simulink model "ForwardKinematic_YuMi"  (R2024a)
(part 20 of 23)

2903273033334964234439083875867/41538374868278621028243970633760768))/10384593717069655257060992658440192 + 34189201462609793352471527538206775118278208232606556159508725/57896044618658097711785492504343953926634992332820282019728792003956564819968))/9007199254740992))/1000 + (2436553109258773196144549622003023*cos(q6R)*(cos(q5R)*((7514214926474921*sin(q4R)*((7514214926474921*cos(q3R)*((7514214926474921*cos(q2R)*((398031123528767*cos(q1R))/562949953421312 - (1392340654334763*sin(q1R))/2251799813685248))/36893488147419103232 - (3480118470877607344838997022995*cos(q2R))/10141204801825835211973625643008 + sin(q2R)*((1392340654334763*cos(q1R))/2251799813685248 + (398031123528767*sin(q1R))/562949953421312)))/36893488147419103232 - sin(q3R)*((3480118470877607344838997022995*sin(q2R))/10141204801825835211973625643008 + cos(q2R)*((1392340654334763*cos(q1R))/2251799813685248 + (398031123528767*sin(q1R))/562949953421312) - (7514214926474921*sin(q2R)*((398031123528767*cos(q1R))/562949953421312 - (1392340654334763*sin(q1R))/2251799813685248))/36893488147419103232) + (9007199067919185*cos(q3R)*((3585145564851136108341178694895*cos(q1R))/5070602400912917605986812821504 - (12541089443950065443620820128155*sin(q1R))/20282409603651670423947251286016 + 2903273033334964234439083875867/41538374868278621028243970633760768))/9007199254740992))/36893488147419103232 + ((7514214926474921*cos(q4R))/36893488147419103232 + (4503599440548691*sin(q4R))/4503599627370496)*(cos(q3R)*((3480118470877607344838997022995*sin(q2R))/10141204801825835211973625643008 + cos(q2R)*((1392340654334763*cos(q1R))/2251799813685248 + (398031123528767*sin(q1R))/562949953421312) - (7514214926474921*sin(q2R)*((398031123528767*cos(q1R))/562949953421312 - (1392340654334763*sin(q1R))/2251799813685248))/36893488147419103232) + (7514214926474921*sin(q3R)*((7514214926474921*cos(q2R)*((398031123528767*cos(q1R))/562949953421312 - (1392340654334763*sin(q1R))/2251799813685248))/36893488147419103232 - (3480118470877607344838997022995*cos(q2R))/10141204801825835211973625643008 + sin(q2R)*((1392340654334763*cos(q1R))/2251799813685248 + (398031123528767*sin(q1R))/562949953421312)))/36893488147419103232 + (9007199067919185*sin(q3R)*((3585145564851136108341178694895*cos(q1R))/5070602400912917605986812821504 - (12541089443950065443620820128155*sin(q1R))/20282409603651670423947251286016 + 2903273033334964234439083875867/41538374868278621028243970633760768))/9007199254740992) - ((9007199067919185*cos(q4R))/9007199254740992 - (234819211581865*sin(q4R))/1152921504606846976)*((26939554316989768830159504461322709929728228295*cos(q1R))/187072209578355573530071658587684226515959365500928 + (31346119847137124244279794758002175024246659075*cos(q2R))/91343852333181432387730302044767688728495783936 - (94236441493986648894942587121893377357613500755*sin(q1R))/748288838313422294120286634350736906063837462003712 - (67682029681889335677290557259385*cos(q2R)*((398031123528767*cos(q1R))/562949953421312 - (1392340654334763*sin(q1R))/2251799813685248))/332306998946228968225951765070086144 - (9007199067919185*sin(q2R)*((1392340654334763*cos(q1R))/2251799813685248 + (398031123528767*sin(q1R))/562949953421312))/9007199254740992 + 21815817562717709140362801846989786744252631507/1532495540865888858358347027150309183618739122183602176)) - (7514214926474921*sin(q5R)*(((4503599440548691*cos(q4R))/4503599627370496 - (7514214926474921*sin(q4R))/36893488147419103232)*(cos(q3R)*((3480118470877607344838997022995*sin(q2R))/10141204801825835211973625643008 + cos(q2R)*((1392340654334763*cos(q1R))/2251799813685248 + (398031123528767*sin(q1R))/562949953421312) - (7514214926474921*sin(q2R)*((398031123528767*cos(q1R))/562949953421312 - (1392340654334763*sin(q1R))/2251799813685248))/36893488147419103232) + (7514214926474921*sin(q3R)*((7514214926474921*cos(q2R)*((398031123528767*cos(q1R))/562949953421312 - (1392340654334763*sin(q1R))/2251799813685248))/36893488147419103232 - (3480118470877607344838997022995*cos(q2R))/10141204801825835211973625643008 + sin(q2R)*((1392340654334763*cos(q1R))/2251799813685248 + (398031123528767*sin(q1R))/562949953421312)))/36893488147419103232 + (9007199067919185*sin(q3R)*((3585145564851136108341178694895*cos(q1R))/5070602400912917605986812821504 - (12541089443950065443620820128155*sin(q1R))/20282409603651670423947251286016 + 2903273033334964234439083875867/41538374868278621028243970633760768))/9007199254740992) + ((234819211581865*cos(q4R))/1152921504606846976 + (9007199067919185*sin(q4R))/9007199254740992)*((26939554316989768830159504461322709929728228295*cos(q1R))/187072209578355573530071658587684226515959365500928 + (31346119847137124244279794758002175024246659075*cos(q2R))/91343852333181432387730302044767688728495783936 - (94236441493986648894942587121893377357613500755*sin(q1R))/748288838313422294120286634350736906063837462003712 - (67682029681889335677290557259385*cos(q2R)*((398031123528767*cos(q1R))/562949953421312 - (1392340654334763*sin(q1R))/2251799813685248))/332306998946228968225951765070086144 - (9007199067919185*sin(q2R)*((1392340654334763*cos(q1R))/2251799813685248 + (398031123528767*sin(q1R))/562949953421312))/9007199254740992 + 21815817562717709140362801846989786744252631507/1532495540865888858358347027150309183618739122183602176) + (7514214926474921*cos(q4R)*((7514214926474921*cos(q3R)*((7514214926474921*cos(q2R)*((398031123528767*cos(q1R))/562949953421312 - (1392340654334763*sin(q1R))/2251799813685248))/36893488147419103232 - (3480118470877607344838997022995*cos(q2R))/10141204801825835211973625643008 + sin(q2R)*((1392340654334763*cos(q1R))/2251799813685248 + (398031123528767*sin(q1R))/562949953421312)))/36893488147419103232 - sin(q3R)*((3480118470877607344838997022995*sin(q2R))/10141204801825835211973625643008 + cos(q2R)*((1392340654334763*cos(q1R))/2251799813685248 + (398031123528767*sin(q1R))/562949953421312) - (7514214926474921*sin(q2R)*((398031123528767*cos(q1R))/562949953421312 - (1392340654334763*sin(q1R))/2251799813685248))/36893488147419103232) + (9007199067919185*cos(q3R)*((3585145564851136108341178694895*cos(q1R))/5070602400912917605986812821504 - (12541089443950065443620820128155*sin(q1R))/20282409603651670423947251286016 + 2903273033334964234439083875867/41538374868278621028243970633760768))/9007199254740992))/36893488147419103232))/36893488147419103232 + (9007199067919185*sin(q5R)*((42218993040650622024393554167529407181397382817729417611526625*cos(q1R))/7067388259113537318333190002971674063309935587502475832486424805170479104 + (49124851885283889459147163519037433596494512994900179139213125*cos(q2R))/3450873173395281893717377931138512726225554486085193277581262111899648 - (147684984717849177105467939785270041851792306559769220895307125*sin(q1R))/28269553036454149273332760011886696253239742350009903329945699220681916416 - (67682029681889335677290557259385*cos(q3R)*((7514214926474921*cos(q2R)*((398031123528767*cos(q1R))/562949953421312 - (1392340654334763*sin(q1R))/2251799813685248))/36893488147419103232 - (3480118470877607344838997022995*cos(q2R))/10141204801825835211973625643008 + sin(q2R)*((1392340654334763*cos(q1R))/2251799813685248 + (398031123528767*sin(q1R))/562949953421312)))/332306998946228968225951765070086144 + (234819211581865*cos(q3R)*((3480118470877607344838997022995*sin(q2R))/10141204801825835211973625643008 + cos(q2R)*((1392340654334763*cos(q1R))/2251799813685248 + (398031123528767*sin(q1R))/562949953421312) - (7514214926474921*sin(q2R)*((398031123528767*cos(q1R))/562949953421312 - (1392340654334763*sin(q1R))/2251799813685248))/36893488147419103232))/1152921504606846976 + (1764482024691522628700660907665*sin(q3R)*((7514214926474921*cos(q2R)*((398031123528767*cos(q1R))/562949953421312 - (1392340654334763*sin(q1R))/2251799813685248))/36893488147419103232 - (3480118470877607344838997022995*cos(q2R))/10141204801825835211973625643008 + sin(q2R)*((1392340654334763*cos(q1R))/2251799813685248 + (398031123528767*sin(q1R))/562949953421312)))/42535295865117307932921825928971026432 + (9007199067919185*sin(q3R)*((3480118470877607344838997022995*sin(q2R))/10141204801825835211973625643008 + cos(q2R)*((1392340654334763*cos(q1R))/2251799813685248 + (398031123528767*sin(q1R))/562949953421312) - (7514214926474921*sin(q2R)*((398031123528767*cos(q1R))/562949953421312 - (1392340654334763*sin(q1R))/2251799813685248))/36893488147419103232))/9007199254740992 - (106069577339469832923929692356850887620017617375*cos(q2R)*((398031123528767*cos(q1R))/562949953421312 - (1392340654334763*sin(q1R))/2251799813685248))/12554203470773361527671578846415332832204710888928069025792 - (81129635049124235038645691064225*cos(q3R)*((3585145564851136108341178694895*cos(q1R))/5070602400912917605986812821504 - (12541089443950065443620820128155*sin(q1R))/20282409603651670423947251286016 + 2903273033334964234439083875867/41538374868278621028243970633760768))/81129638414606681695789005144064 - (14115856197532180673579726082375*sin(q2R)*((1392340654334763*cos(q1R))/2251799813685248 + (398031123528767*sin(q1R))/562949953421312))/340282366920938463463374607431768211456 + (2115063383689692319117831580025*sin(q3R)*((3585145564851136108341178694895*cos(q1R))/5070602400912917605986812821504 - (12541089443950065443620820128155*sin(q1R))/20282409603651670423947251286016 + 2903273033334964234439083875867/41538374868278621028243970633760768))/10384593717069655257060992658440192 + 34189201462609793352471527538206775118278208232606556159508725/57896044618658097711785492504343953926634992332820282019728792003956564819968))/9007199254740992))/332306998946228968225951765070086144000 + (324259171862923063*sin(q6R)*((7514214926474921*cos(q5R)*(((4503599440548691*cos(q4R))/4503599627370496 - (7514214926474921*sin(q4R))/36893488147419103232)*(cos(q3R)*((3480118470877607344838997022995*sin(q2R))/10141204801825835211973625643008 + cos(q2R)*((1392340654334763*cos(q1R))/2251799813685248 + (398031123528767*sin(q1R))/562949953421312) - (7514214926474921*sin(q2R)*((398031123528767*cos(q1R))/562949953421312 - (1392340654334763*sin(q1R))/2251799813685248))/36893488147419103232) + (7514214926474921*sin(q3R)*((7514214926474921*cos(q2R)*((398031123528767*cos(q1R))/562949953421312 - (1392340654334763*sin(q1R))/2251799813685248))/36893488147419103232 - (3480118470877607344838997022995*cos(q2R))/10141204801825835211973625643008 + sin(q2R)*((1392340654334763*cos(q1R))/2251799813685248 + (398031123528767*sin(q1R))/562949953421312)))/36893488147419103232 + (9007199067919185*sin(q3R)*((3585145564851136108341178694895*cos(q1R))/5070602400912917605986812821504 - (12541089443950065443620820128155*sin(q1R))/20282409603651670423947251286016 + 2903273033334964234439083875867/41538374868278621028243970633760768))/9007199254740992) + ((234819211581865*cos(q4R))/1152921504606846976 + (9007199067919185*sin(q4R))/9007199254740992)*((26939554316989768830159504461322709929728228295*cos(q1R))/187072209578355573530071658587684226515959365500928 + (31346119847137124244279794758002175024246659075*cos(q2R))/91343852333181432387730302044767688728495783936 - (94236441493986648894942587121893377357613500755*sin(q1R))/748288838313422294120286634350736906063837462003712 - (67682029681889335677290557259385*cos(q2R)*((398031123528767*cos(q1R))/562949953421312 - (1392340654334763*sin(q1R))/2251799813685248))/332306998946228968225951765070086144 - (9007199067919185*sin(q2R)*((1392340654334763*cos(q1R))/2251799813685248 + (398031123528767*sin(q1R))/562949953421312))/9007199254740992 + 21815817562717709140362801846989786744252631507/1532495540865888858358347027150309183618739122183602176) + (7514214926474921*cos(q4R)*((7514214926474921*cos(q3R)*((7514214926474921*cos(q2R)*((398031123528767*cos(q1R))/562949953421312 - (1392340654334763*sin(q1R))/2251799813685248))/36893488147419103232 - (3480118470877607344838997022995*cos(q2R))/10141204801825835211973625643008 + sin(q2R)*((1392340654334763*cos(q1R))/2251799813685248 + (398031123528767*sin(q1R))/562949953421312)))/36893488147419103232 - sin(q3R)*((3480118470877607344838997022995*sin(q2R))/10141204801825835211973625643008 + cos(q2R)*((1392340654334763*cos(q1R))/2251799813685248 + (398031123528767*sin(q1R))/562949953421312) - (7514214926474921*sin(q2R)*((398031123528767*cos(q1R))/562949953421312 - (1392340654334763*sin(q1R))/2251799813685248))/36893488147419103232) + (9007199067919185*cos(q3R)*((3585145564851136108341178694895*cos(q1R))/5070602400912917605986812821504 - (12541089443950065443620820128155*sin(q1R))/20282409603651670423947251286016 + 2903273033334964234439083875867/41538374868278621028243970633760768))/9007199254740992))/36893488147419103232))/36893488147419103232 + sin(q5R)*((7514214926474921*sin(q4R)*((7514214926474921*cos(q3R)*((7514214926474921*cos(q2R)*((398031123528767*cos(q1R))/562949953421312 - (1392340654334763*sin(q1R))/2251799813685248))/36893488147419103232 - (3480118470877607344838997022995*cos(q2R))/10141204801825835211973625643008 + sin(q2R)*((1392340654334763*cos(q1R))/2251799813685248 + (398031123528767*sin(q1R))/562949953421312)))/36893488147419103232 - sin(q3R)*((3480118470877607344838997022995*sin(q2R))/10141204801825835211973625643008 + cos(q2R)*((1392340654334763*cos(q1R))/2251799813685248 + (398031123528767*sin(q1R))/562949953421312) - (7514214926474921*sin(q2R)*((398031123528767*cos(q1R))/562949953421312 - (1392340654334763*sin(q1R))/2251799813685248))/36893488147419103232) + (9007199067919185*cos(q3R)*((3585145564851136108341178694895*cos(q1R))/5070602400912917605986812821504 - (12541089443950065443620820128155*sin(q1R))/20282409603651670423947251286016 + 2903273033334964234439083875867/41538374868278621028243970633760768))/9007199254740992))/36893488147419103232 + ((7514214926474921*cos(q4R))/36893488147419103232 + (4503599440548691*sin(q4R))/4503599627370496)*(cos(q3R)*((3480118470877607344838997022995*sin(q2R))/10141204801825835211973625643008 + cos(q2R)*((1392340654334763*cos(q1R))/2251799813685248 + (398031123528767*sin(q1R))/562949953421312) - (7514214926474921*sin(q2R)*((398031123528767*cos(q1R))/562949953421312 - (1392340654334763*sin(q1R))/2251799813685248))/36893488147419103232) + (7514214926474921*sin(q3R)*((7514214926474921*cos(q2R)*((398031123528767*cos(q1R))/562949953421312 - (1392340654334763*sin(q1R))/2251799813685248))/36893488147419103232 - (3480118470877607344838997022995*cos(q2R))/10141204801825835211973625643008 + sin(q2R)*((1392340654334763*cos(q1R))/2251799813685248 + (398031123528767*sin(q1R))/562949953421312)))/36893488147419103232 + (9007199067919185*sin(q3R)*((3585145564851136108341178694895*cos(q1R))/5070602400912917605986812821504 - (12541089443950065443620820128155*sin(q1R))/20282409603651670423947251286016 + 2903273033334964234439083875867/41538374868278621028243970633760768))/9007199254740992) - ((9007199067919185*cos(q4R))/9007199254740992 - (234819211581865*sin(q4R))/1152921504606846976)*((26939554316989768830159504461322709929728228295*cos(q1R))/187072209578355573530071658587684226515959365500928 + (31346119847137124244279794758002175024246659075*cos(q2R))/91343852333181432387730302044767688728495783936 - (94236441493986648894942587121893377357613500755*sin(q1R))/748288838313422294120286634350736906063837462003712 - (67682029681889335677290557259385*cos(q2R)*((398031123528767*cos(q1R))/562949953421312 - (1392340654334763*sin(q1R))/2251799813685248))/332306998946228968225951765070086144 - (9007199067919185*sin(q2R)*((1392340654334763*cos(q1R))/2251799813685248 + (398031123528767*sin(q1R))/562949953421312))/9007199254740992 + 21815817562717709140362801846989786744252631507/1532495540865888858358347027150309183618739122183602176)) - (9007199067919185*cos(q5R)*((42218993040650622024393554167529407181397382817729417611526625*cos(q1R))/7067388259113537318333190002971674063309935587502475832486424805170479104 + (49124851885283889459147163519037433596494512994900179139213125*cos(q2R))/3450873173395281893717377931138512726225554486085193277581262111899648 - (147684984717849177105467939785270041851792306559769220895307125*sin(q1R))/28269553036454149273332760011886696253239742350009903329945699220681916416 - (67682029681889335677290557259385*cos(q3R)*((7514214926474921*cos(q2R)*((398031123528767*cos(q1R))/562949953421312 - (1392340654334763*sin(q1R))/2251799813685248))/36893488147419103232 - (3480118470877607344838997022995*cos(q2R))/10141204801825835211973625643008 + sin(q2R)*((1392340654334763*cos(q1R))/2251799813685248 + (398031123528767*sin(q1R))/562949953421312)))/332306998946228968225951765070086144 + (234819211581865*cos(q3R)*((3480118470877607344838997022995*sin(q2R))/10141204801825835211973625643008 + cos(q2R)*((1392340654334763*cos(q1R))/2251799813685248 + (398031123528767*sin(q1R))/562949953421312) - (7514214926474921*sin(q2R)*((398031123528767*cos(q1R))/562949953421312 - (1392340654334763*sin(q1R))/2251799813685248))/36893488147419103232))/1152921504606846976 + (1764482024691522628700660907665*sin(q3R)*((7514214926474921*cos(q2R)*((398031123528767*cos(q1R))/562949953421312 - (1392340654334763*sin(q1R))/2251799813685248))/36893488147419103232 - (3480118470877607344838997022995*cos(q2R))/10141204801825835211973625643008 + sin(q2R)*((1392340654334763*cos(q1R))/2251799813685248 + (398031123528767*sin(q1R))/562949953421312)))/42535295865117307932921825928971026432 + (9007199067919185*sin(q3R)*((3480118470877607344838997022995*sin(q2R))/10141204801825835211973625643008 + cos(q2R)*((1392340654334763*cos(q1R))/2251799813685248 + (398031123528767*sin(q1R))/562949953421312) - (7514214926474921*sin(q2R)*((398031123528767*cos(q1R))/562949953421312 - (1392340654334763*sin(q1R))/2251799813685248))/36893488147419103232))/9007199254740992 - (106069577339469832923929692356850887620017617375*cos(q2R)*((398031123528767*cos(q1R))/562949953421312 - (1392340654334763*sin(q1R))/2251799813685248))/12554203470773361527671578846415332832204710888928069025792 - (81129635049124235038645691064225*cos(q3R)*((3585145564851136108341178694895*cos(q1R))/5070602400912917605986812821504 - (12541089443950065443620820128155*sin(q1R))/20282409603651670423947251286016 + 2903273033334964234439083875867/41538374868278621028243970633760768))/81129638414606681695789005144064 - (14115856197532180673579726082375*sin(q2R)*((1392340654334763*cos(q1R))/2251799813685248 + (398031123528767*sin(q1R))/562949953421312))/340282366920938463463374607431768211456 + (2115063383689692319117831580025*sin(q3R)*((3585145564851136108341178694895*cos(q1R))/5070602400912917605986812821504 - (12541089443950065443620820128155*sin(q1R))/20282409603651670423947251286016 + 2903273033334964234439083875867/41538374868278621028243970633760768))/10384593717069655257060992658440192 + 34189201462609793352471527538206775118278208232606556159508725/57896044618658097711785492504343953926634992332820282019728792003956564819968))/9007199254740992))/9007199254740992000 + (712008244765680093343103025701132101054572137019*sin(q5R)*(((4503599440548691*cos(q4R))/4503599627370496 - (7514214926474921*sin(q4R))/36893488147419103232)*(cos(q3R)*((3480118470877607344838997022995*sin(q2R))/10141204801825835211973625643008 + cos(q2R)*((1392340654334763*cos(q1R))/2251799813685248 + (398031123528767*sin(q1R))/562949953421312) - (7514214926474921*sin(q2R)*((398031123528767*cos(q1R))/562949953421312 - (1392340654334763*sin(q1R))/2251799813685248))/36893488147419103232) + (7514214926474921*sin(q3R)*((7514214926474921*cos(q2R)*((398031123528767*cos(q1R))/562949953421312 - (1392340654334763*sin(q1R))/2251799813685248))/36893488147419103232 - (3480118470877607344838997022995*cos(q2R))/10141204801825835211973625643008 + sin(q2R)*((1392340654334763*cos(q1R))/2251799813685248 + (398031123528767*sin(q1R))/562949953421312)))/36893488147419103232 + (9007199067919185*sin(q3R)*((3585145564851136108341178694895*cos(q1R))/5070602400912917605986812821504 - (12541089443950065443620820128155*sin(q1R))/20282409603651670423947251286016 + 2903273033334964234439083875867/41538374868278621028243970633760768))/9007199254740992) + ((234819211581865*cos(q4R))/1152921504606846976 + (9007199067919185*sin(q4R))/9007199254740992)*((26939554316989768830159504461322709929728228295*cos(q1R))/187072209578355573530071658587684226515959365500928 + (31346119847137124244279794758002175024246659075*cos(q2R))/91343852333181432387730302044767688728495783936 - (94236441493986648894942587121893377357613500755*sin(q1R))/748288838313422294120286634350736906063837462003712 - (67682029681889335677290557259385*cos(q2R)*((398031123528767*cos(q1R))/562949953421312 - (1392340654334763*sin(q1R))/2251799813685248))/332306998946228968225951765070086144 - (9007199067919185*sin(q2R)*((1392340654334763*cos(q1R))/2251799813685248 + (398031123528767*sin(q1R))/562949953421312))/9007199254740992 + 21815817562717709140362801846989786744252631507/1532495540865888858358347027150309183618739122183602176) + (7514214926474921*cos(q4R)*((7514214926474921*cos(q3R)*((7514214926474921*cos(q2R)*((398031123528767*cos(q1R))/562949953421312 - (1392340654334763*sin(q1R))/2251799813685248))/36893488147419103232 - (3480118470877607344838997022995*cos(q2R))/10141204801825835211973625643008 + sin(q2R)*((1392340654334763*cos(q1R))/2251799813685248 + (398031123528767*sin(q1R))/562949953421312)))/36893488147419103232 - sin(q3R)*((3480118470877607344838997022995*sin(q2R))/10141204801825835211973625643008 + cos(q2R)*((1392340654334763*cos(q1R))/2251799813685248 + (398031123528767*sin(q1R))/562949953421312) - (7514214926474921*sin(q2R)*((398031123528767*cos(q1R))/562949953421312 - (1392340654334763*sin(q1R))/2251799813685248))/36893488147419103232) + (9007199067919185*cos(q3R)*((3585145564851136108341178694895*cos(q1R))/5070602400912917605986812821504 - (12541089443950065443620820128155*sin(q1R))/20282409603651670423947251286016 + 2903273033334964234439083875867/41538374868278621028243970633760768))/9007199254740992))/36893488147419103232))/2451992865385422173373355243440494693789982595493763481600 - (94754841554645069948206780163139*cos(q5R)*((7514214926474921*sin(q4R)*((7514214926474921*cos(q3R)*((7514214926474921*cos(q2R)*((398031123528767*cos(q1R))/562949953421312 - (1392340654334763*sin(q1R))/2251799813685248))/36893488147419103232 - (3480118470877607344838997022995*cos(q2R))/10141204801825835211973625643008 + sin(q2R)*((1392340654334763*cos(q1R))/2251799813685248 + (398031123528767*sin(q1R))/562949953421312)))/36893488147419103232 - sin(q3R)*((3480118470877607344838997022995*sin(q2R))/10141204801825835211973625643008 + cos(q2R)*((1392340654334763*cos(q1R))/2251799813685248 + (398031123528767*sin(q1R))/562949953421312) - (7514214926474921*sin(q2R)*((398031123528767*cos(q1R))/562949953421312 - (1392340654334763*sin(q1R))/2251799813685248))/36893488147419103232) + (9007199067919185*cos(q3R)*((3585145564851136108341178694895*cos(q1R))/5070602400912917605986812821504 - (12541089443950065443620820128155*sin(q1R))/20282409603651670423947251286016 + 2903273033334964234439083875867/41538374868278621028243970633760768))/9007199254740992))/36893488147419103232 + ((7514214926474921*cos(q4R))/36893488147419103232 + (4503599440548691*sin(q4R))/4503599627370496)*(cos(q3R)*((3480118470877607344838997022995*sin(q2R))/10141204801825835211973625643008 + cos(q2R)*((1392340654334763*cos(q1R))/2251799813685248 + (398031123528767*sin(q1R))/562949953421312) - (7514214926474921*sin(q2R)*((398031123528767*cos(q1R))/562949953421312 - (1392340654334763*sin(q1R))/2251799813685248))/36893488147419103232) + (7514214926474921*sin(q3R)*((7514214926474921*cos(q2R)*((398031123528767*cos(q1R))/562949953421312 - (1392340654334763*sin(q1R))/2251799813685248))/36893488147419103232 - (3480118470877607344838997022995*cos(q2R))/10141204801825835211973625643008 + sin(q2R)*((1392340654334763*cos(q1R))/2251799813685248 + (398031123528767*sin(q1R))/562949953421312)))/36893488147419103232 + (9007199067919185*sin(q3R)*((3585145564851136108341178694895*cos(q1R))/5070602400912917605986812821504 - (12541089443950065443620820128155*sin(q1R))/20282409603651670423947251286016 + 2903273033334964234439083875867/41538374868278621028243970633760768))/9007199254740992) - ((9007199067919185*cos(q4R))/9007199254740992 - (234819211581865*sin(q4R))/1152921504606846976)*((26939554316989768830159504461322709929728228295*cos(q1R))/187072209578355573530071658587684226515959365500928 + (31346119847137124244279794758002175024246659075*cos(q2R))/91343852333181432387730302044767688728495783936 - (94236441493986648894942587121893377357613500755*sin(q1R))/748288838313422294120286634350736906063837462003712 - (67682029681889335677290557259385*cos(q2R)*((398031123528767*cos(q1R))/562949953421312 - (1392340654334763*sin(q1R))/2251799813685248))/332306998946228968225951765070086144 - (9007199067919185*sin(q2R)*((1392340654334763*cos(q1R))/2251799813685248 + (398031123528767*sin(q1R))/562949953421312))/9007199254740992 + 21815817562717709140362801846989786744252631507/1532495540865888858358347027150309183618739122183602176)))/66461399789245793645190353014017228800 + (202883803014822867*sin(q6R)*(cos(q5R)*((7514214926474921*sin(q4R)*((7514214926474921*cos(q3R)*((7514214926474921*cos(q2R)*((398031123528767*cos(q1R))/562949953421312 - (1392340654334763*sin(q1R))/2251799813685248))/36893488147419103232 - (3480118470877607344838997022995*cos(q2R))/10141204801825835211973625643008 + sin(q2R)*((1392340654334763*cos(q1R))/2251799813685248 + (398031123528767*sin(q1R))/562949953421312)))/36893488147419103232 - sin(q3R)*((3480118470877607344838997022995*sin(q2R))/10141204801825835211973625643008 + cos(q2R)*((1392340654334763*cos(q1R))/2251799813685248 + (398031123528767*sin(q1R))/562949953421312) - (7514214926474921*sin(q2R)*((398031123528767*cos(q1R))/562949953421312 - (1392340654334763*sin(q1R))/2251799813685248))/36893488147419103232) + (9007199067919185*cos(q3R)*((3585145564851136108341178694895*cos(q1R))/5070602400912917605986812821504 - (12541089443950065443620820128155*sin(q1R))/20282409603651670423947251286016 + 2903273033334964234439083875867/41538374868278621028243970633760768))/9007199254740992))/36893488147419103232 + ((7514214926474921*cos(q4R))/36893488147419103232 + (4503599440548691*sin(q4R))/4503599627370496)*(cos(q3R)*((3480118470877607344838997022995*sin(q2R))/10141204801825835211973625643008 + cos(q2R)*((1392340654334763*cos(q1R))/2251799813685248 + (398031123528767*sin(q1R))/562949953421312) - (7514214926474921*sin(q2R)*((398031123528767*cos(q1R))/562949953421312 - (1392340654334763*sin(q1R))/2251799813685248))/36893488147419103232) + (7514214926474921*sin(q3R)*((7514214926474921*cos(q2R)*((398031123528767*cos(q1R))/562949953421312 - (1392340654334763*sin(q1R))/2251799813685248))/36893488147419103232 - (3480118470877607344838997022995*cos(q2R))/10141204801825835211973625643008 + sin(q2R)*((1392340654334763*cos(q1R))/2251799813685248 + (398031123528767*sin(q1R))/562949953421312)))/36893488147419103232 + (9007199067919185*sin(q3R)*((3585145564851136108341178694895*cos(q1R))/5070602400912917605986812821504 - (12541089443950065443620820128155*sin(q1R))/20282409603651670423947251286016 + 2903273033334964234439083875867/41538374868278621028243970633760768))/9007199254740992) - ((9007199067919185*cos(q4R))/9007199254740992 - (234819211581865*sin(q4R))/1152921504606846976)*((26939554316989768830159504461322709929728228295*cos(q1R))/187072209578355573530071658587684226515959365500928 + (31346119847137124244279794758002175024246659075*cos(q2R))/91343852333181432387730302044767688728495783936 - (94236441493986648894942587121893377357613500755*sin(q1R))/748288838313422294120286634350736906063837462003712 - (67682029681889335677290557259385*cos(q2R)*((398031123528767*cos(q1R))/562949953421312 - (1392340654334763*sin(q1R))/2251799813685248))/332306998946228968225951765070086144 - (9007199067919185*sin(q2R)*((1392340654334763*cos(q1R))/2251799813685248 + (398031123528767*sin(q1R))/562949953421312))/9007199254740992 + 21815817562717709140362801846989786744252631507/1532495540865888858358347027150309183618739122183602176)) - (7514214926474921*sin(q5R)*(((4503599440548691*cos(q4R))/4503599627370496 - (7514214926474921*sin(q4R))/36893488147419103232)*(cos(q3R)*((3480118470877607344838997022995*sin(q2R))/10141204801825835211973625643008 + cos(q2R)*((1392340654334763*cos(q1R))/2251799813685248 + (398031123528767*sin(q1R))/562949953421312) - (7514214926474921*sin(q2R)*((398031123528767*cos(q1R))/562949953421312 - (1392340654334763*sin(q1R))/2251799813685248))/36893488147419103232) + (7514214926474921*sin(q3R)*((7514214926474921*cos(q2R)*((398031123528767*cos(q1R))/562949953421312 - (1392340654334763*sin(q1R))/2251799813685248))/36893488147419103232 - (3480118470877607344838997022995*cos(q2R))/10141204801825835211973625643008 + sin(q2R)*((1392340654334763*cos(q1R))/2251799813685248 + (398031123528767*sin(q1R))/562949953421312)))/36893488147419103232 + (9007199067919185*sin(q3R)*((3585145564851136108341178694895*cos(q1R))/5070602400912917605986812821504 - (12541089443950065443620820128155*sin(q1R))/20282409603651670423947251286016 + 2903273033334964234439083875867/41538374868278621028243970633760768))/9007199254740992) + ((234819211581865*cos(q4R))/1152921504606846976 + (9007199067919185*sin(q4R))/9007199254740992)*((26939554316989768830159504461322709929728228295*cos(q1R))/187072209578355573530071658587684226515959365500928 + (31346119847137124244279794758002175024246659075*cos(q2R))/91343852333181432387730302044767688728495783936 - (94236441493986648894942587121893377357613500755*sin(q1R))/748288838313422294120286634350736906063837462003712 - (67682029681889335677290557259385*cos(q2R)*((398031123528767*cos(q1R))/562949953421312 - (1392340654334763*sin(q1R))/2251799813685248))/332306998946228968225951765070086144 - (9007199067919185*sin(q2R)*((1392340654334763*cos(q1R))/2251799813685248 + (398031123528767*sin(q1R))/562949953421312))/9007199254740992 + 21815817562717709140362801846989786744252631507/1532495540865888858358347027150309183618739122183602176) + (7514214926474921*cos(q4R)*((7514214926474921*cos(q3R)*((7514214926474921*cos(q2R)*((398031123528767*cos(q1R))/562949953421312 - (1392340654334763*sin(q1R))/2251799813685248))/36893488147419103232 - (3480118470877607344838997022995*cos(q2R))/10141204801825835211973625643008 + sin(q2R)*((1392340654334763*cos(q1R))/2251799813685248 + (398031123528767*sin(q1R))/562949953421312)))/36893488147419103232 - sin(q3R)*((3480118470877607344838997022995*sin(q2R))/10141204801825835211973625643008 + cos(q2R)*((1392340654334763*cos(q1R))/2251799813685248 + (398031123528767*sin(q1R))/562949953421312) - (7514214926474921*sin(q2R)*((398031123528767*cos(q1R))/562949953421312 - (1392340654334763*sin(q1R))/2251799813685248))/36893488147419103232) + (9007199067919185*cos(q3R)*((3585145564851136108341178694895*cos(q1R))/5070602400912917605986812821504 - (12541089443950065443620820128155*sin(q1R))/20282409603651670423947251286016 + 2903273033334964234439083875867/41538374868278621028243970633760768))/9007199254740992))/36893488147419103232))/36893488147419103232 + (9007199067919185*sin(q5R)*((42218993040650622024393554167529407181397382817729417611526625*cos(q1R))/7067388259113537318333190002971674063309935587502475832486424805170479104 + (49124851885283889459147163519037433596494512994900179139213125*cos(q2R))/3450873173395281893717377931138512726225554486085193277581262111899648 - (147684984717849177105467939785270041851792306559769220895307125*sin(q1R))/28269553036454149273332760011886696253239742350009903329945699220681916416 - (67682029681889335677290557259385*cos(q3R)*((7514214926474921*cos(q2R)*((398031123528767*cos(q1R))/562949953421312 - (1392340654334763*sin(q1R))/2251799813685248))/36893488147419103232 - (3480118470877607344838997022995*cos(q2R))/10141204801825835211973625643008 + sin(q2R)*((1392340654334763*cos(q1R))/2251799813685248 + (398031123528767*sin(q1R))/562949953421312)))/332306998946228968225951765070086144 + (234819211581865*cos(q3R)*((3480118470877607344838997022995*sin(q2R))/10141204801825835211973625643008 + cos(q2R)*((1392340654334763*cos(q1R))/2251799813685248 + (398031123528767*sin(q1R))/562949953421312) - (7514214926474921*sin(q2R)*((398031123528767*cos(q1R))/562949953421312 - (1392340654334763*sin(q1R))/2251799813685248))/36893488147419103232))/1152921504606846976 + (1764482024691522628700660907665*sin(q3R)*((7514214926474921*cos(q2R)*((398031123528767*cos(q1R))/562949953421312 - (1392340654334763*sin(q1R))/2251799813685248))/36893488147419103232 - (3480118470877607344838997022995*cos(q2R))/10141204801825835211973625643008 + sin(q2R)*((1392340654334763*cos(q1R))/2251799813685248 + (398031123528767*sin(q1R))/562949953421312)))/42535295865117307932921825928971026432 + (9007199067919185*sin(q3R)*((3480118470877607344838997022995*sin(q2R))/10141204801825835211973625643008 + cos(q2R)*((1392340654334763*cos(q1R))/2251799813685248 + (398031123528767*sin(q1R))/562949953421312) - (7514214926474921*sin(q2R)*((398031123528767*cos(q1R))/562949953421312 - (1392340654334763*sin(q1R))/2251799813685248))/36893488147419103232))/9007199254740992 - (106069577339469832923929692356850887620017617375*cos(q2R)*((398031123528767*cos(q1R))/562949953421312 - (1392340654334763*sin(q1R))/2251799813685248))/12554203470773361527671578846415332832204710888928069025792 - (81129635049124235038645691064225*cos(q3R)*((3585145564851136108341178694895*cos(q1R))/5070602400912917605986812821504 - (12541089443950065443620820128155*sin(q1R))/20282409603651670423947251286016 + 2903273033334964234439083875867/41538374868278621028243970633760768))/81129638414606681695789005144064 - (14115856197532180673579726082375*sin(q2R)*((1392340654334763*cos(q1R))/2251799813685248 + (398031123528767*sin(q1R))/562949953421312))/340282366920938463463374607431768211456 + (2115063383689692319117831580025*sin(q3R)*((3585145564851136108341178694895*cos(q1R))/5070602400912917605986812821504 - (12541089443950065443620820128155*sin(q1R))/20282409603651670423947251286016 + 2903273033334964234439083875867/41538374868278621028243970633760768))/10384593717069655257060992658440192 + 34189201462609793352471527538206775118278208232606556159508725/57896044618658097711785492504343953926634992332820282019728792003956564819968))/9007199254740992))/36893488147419103232000 + (27*sin(q5R)*((7514214926474921*sin(q4R)*((7514214926474921*cos(q3R)*((7514214926474921*cos(q2R)*((398031123528767*cos(q1R))/562949953421312 - (1392340654334763*sin(q1R))/2251799813685248))/36893488147419103232 - (3480118470877607344838997022995*cos(q2R))/10141204801825835211973625643008 + sin(q2R)*((1392340654334763*cos(q1R))/2251799813685248 + (398031123528767*sin(q1R))/562949953421312)))/36893488147419103232 - sin(q3R)*((3480118470877607344838997022995*sin(q2R))/10141204801825835211973625643008 + cos(q2R)*((1392340654334763*cos(q1R))/2251799813685248 + (398031123528767*sin(q1R))/562949953421312) - (7514214926474921*sin(q2R)*((398031123528767*cos(q1R))/562949953421312 - (1392340654334763*sin(q1R))/2251799813685248))/36893488147419103232) + (9007199067919185*cos(q3R)*((3585145564851136108341178694895*cos(q1R))/5070602400912917605986812821504 - (12541089443950065443620820128155*sin(q1R))/20282409603651670423947251286016 + 2903273033334964234439083875867/41538374868278621028243970633760768))/9007199254740992))/36893488147419103232 + ((7514214926474921*cos(q4R))/36893488147419103232 + (4503599440548691*sin(q4R))/4503599627370496)*(cos(q3R)*((3480118470877607344838997022995*sin(q2R))/10141204801825835211973625643008 + cos(q2R)*((1392340654334763*cos(q1R))/2251799813685248 + (398031123528767*sin(q1R))/562949953421312) - (7514214926474921*sin(q2R)*((398031123528767*cos(q1R))/562949953421312 - (1392340654334763*sin(q1R))/2251799813685248))/36893488147419103232) + (7514214926474921*sin(q3R)*((7514214926474921*cos(q2R)*((398031123528767*cos(q1R))/562949953421312 - (1392340654334763*sin(q1R))/2251799813685248))/36893488147419103232 - (3480118470877607344838997022995*cos(q2R))/10141204801825835211973625643008 + sin(q2R)*((1392340654334763*cos(q1R))/2251799813685248 + (398031123528767*sin(q1R))/562949953421312)))/36893488147419103232 + (9007199067919185*sin(q3R)*((3585145564851136108341178694895*cos(q1R))/5070602400912917605986812821504 - (12541089443950065443620820128155*sin(q1R))/20282409603651670423947251286016 + 2903273033334964234439083875867/41538374868278621028243970633760768))/9007199254740992) - ((9007199067919185*cos(q4R))/9007199254740992 - (234819211581865*sin(q4R))/1152921504606846976)*((26939554316989768830159504461322709929728228295*cos(q1R))/187072209578355573530071658587684226515959365500928 + (31346119847137124244279794758002175024246659075*cos(q2R))/91343852333181432387730302044767688728495783936 - (94236441493986648894942587121893377357613500755*sin(q1R))/748288838313422294120286634350736906063837462003712 - (67682029681889335677290557259385*cos(q2R)*((398031123528767*cos(q1R))/562949953421312 - (1392340654334763*sin(q1R))/2251799813685248))/332306998946228968225951765070086144 - (9007199067919185*sin(q2R)*((1392340654334763*cos(q1R))/2251799813685248 + (398031123528767*sin(q1R))/562949953421312))/9007199254740992 + 21815817562717709140362801846989786744252631507/1532495540865888858358347027150309183618739122183602176)))/1000 - (48638874966763599*cos(q5R)*((42218993040650622024393554167529407181397382817729417611526625*cos(q1R))/7067388259113537318333190002971674063309935587502475832486424805170479104 + (49124851885283889459147163519037433596494512994900179139213125*cos(q2R))/3450873173395281893717377931138512726225554486085193277581262111899648 - (147684984717849177105467939785270041851792306559769220895307125*sin(q1R))/28269553036454149273332760011886696253239742350009903329945699220681916416 - (67682029681889335677290557259385*cos(q3R)*((7514214926474921*cos(q2R)*((398031123528767*cos(q1R))/562949953421312 - (1392340654334763*sin(q1R))/2251799813685248))/36893488147419103232 - (3480118470877607344838997022995*cos(q2R))/10141204801825835211973625643008 + sin(q2R)*((1392340654334763*cos(q1R))/2251799813685248 + (398031123528767*sin(q1R))/562949953421312)))/332306998946228968225951765070086144 + (234819211581865*cos(q3R)*((3480118470877607344838997022995*sin(q2R))/10141204801825835211973625643008 + cos(q2R)*((1392340654334763*cos(q1R))/2251799813685248 + (398031123528767*sin(q1R))/562949953421312) - (7514214926474921*sin(q2R)*((398031123528767*cos(q1R))/562949953421312 - (1392340654334763*sin(q1R))/2251799813685248))/36893488147419103232))/1152921504606846976 + (1764482024691522628700660907665*sin(q3R)*((7514214926474921*cos(q2R)*((398031123528767*cos(q1R))/562949953421312 - (1392340654334763*sin(q1R))/2251799813685248))/36893488147419103232 - (3480118470877607344838997022995*cos(q2R))/10141204801825835211973625643008 + sin(q2R)*((1392340654334763*cos(q1R))/2251799813685248 + (398031123528767*sin(q1R))/562949953421312)))/42535295865117307932921825928971026432 + (9007199067919185*sin(q3R)*((3480118470877607344838997022995*sin(q2R))/10141204801825835211973625643008 + cos(q2R)*((1392340654334763*cos(q1R))/2251799813685248 + (398031123528767*sin(q1R))/562949953421312) - (7514214926474921*sin(q2R)*((398031123528767*cos(q1R))/562949953421312 - (1392340654334763*sin(q1R))/2251799813685248))/36893488147419103232))/9007199254740992 - (106069577339469832923929692356850887620017617375*cos(q2R)*((398031123528767*cos(q1R))/562949953421312 - (1392340654334763*sin(q1R))/2251799813685248))/12554203470773361527671578846415332832204710888928069025792 - (81129635049124235038645691064225*cos(q3R)*((3585145564851136108341178694895*cos(q1R))/5070602400912917605986812821504 - (12541089443950065443620820128155*sin(q1R))/20282409603651670423947251286016 + 2903273033334964234439083875867/41538374868278621028243970633760768))/81129638414606681695789005144064 - (14115856197532180673579726082375*sin(q2R)*((1392340654334763*cos(q1R))/2251799813685248 + (398031123528767*sin(q1R))/562949953421312))/340282366920938463463374607431768211456 + (2115063383689692319117831580025*sin(q3R)*((3585145564851136108341178694895*cos(q1R))/5070602400912917605986812821504 - (12541089443950065443620820128155*sin(q1R))/20282409603651670423947251286016 + 2903273033334964234439083875867/41538374868278621028243970633760768))/10384593717069655257060992658440192 + 34189201462609793352471527538206775118278208232606556159508725/57896044618658097711785492504343953926634992332820282019728792003956564819968))/1801439850948198400 - (170695144106365826517608855445768431563113584343*sin(q5R)*((42218993040650622024393554167529407181397382817729417611526625*cos(q1R))/7067388259113537318333190002971674063309935587502475832486424805170479104 + (49124851885283889459147163519037433596494512994900179139213125*cos(q2R))/3450873173395281893717377931138512726225554486085193277581262111899648 - (147684984717849177105467939785270041851792306559769220895307125*sin(q1R))/28269553036454149273332760011886696253239742350009903329945699220681916416 - (67682029681889335677290557259385*cos(q3R)*((7514214926474921*cos(q2R)*((398031123528767*cos(q1R))/562949953421312 - (1392340654334763*sin(q1R))/2251799813685248))/36893488147419103232 - (3480118470877607344838997022995*cos(q2R))/10141204801825835211973625643008 + sin(q2R)*((1392340654334763*cos(q1R))/2251799813685248 + (398031123528767*sin(q1R))/562949953421312)))/332306998946228968225951765070086144 + (234819211581865*cos(q3R)*((3480118470877607344838997022995*sin(q2R))/10141204801825835211973625643008 + cos(q2R)*((1392340654334763*cos(q1R))/2251799813685248 + (398031123528767*sin(q1R))/562949953421312) - (7514214926474921*sin(q2R)*((398031123528767*cos(q1R))/562949953421312 - (1392340654334763*sin(q1R))/2251799813685248))/36893488147419103232))/1152921504606846976 + (1764482024691522628700660907665*sin(q3R)*((7514214926474921*cos(q2R)*((398031123528767*cos(q1R))/562949953421312 - (1392340654334763*sin(q1R))/2251799813685248))/36893488147419103232 - (3480118470877607344838997022995*cos(q2R))/10141204801825835211973625643008 + sin(q2R)*((1392340654334763*cos(q1R))/2251799813685248 + (398031123528767*sin(q1R))/562949953421312)))/42535295865117307932921825928971026432 + (9007199067919185*sin(q3R)*((3480118470877607344838997022995*sin(q2R))/10141204801825835211973625643008 + cos(q2R)*((1392340654334763*cos(q1R))/2251799813685248 + (398031123528767*sin(q1R))/562949953421312) - (7514214926474921*sin(q2R)*((398031123528767*cos(q1R))/562949953421312 - (1392340654334763*sin(q1R))/2251799813685248))/36893488147419103232))/9007199254740992 - (106069577339469832923929692356850887620017617375*cos(q2R)*((398031123528767*cos(q1R))/562949953421312 - (1392340654334763*sin(q1R))/2251799813685248))/12554203470773361527671578846415332832204710888928069025792 - (81129635049124235038645691064225*cos(q3R)*((3585145564851136108341178694895*cos(q1R))/5070602400912917605986812821504 - (12541089443950065443620820128155*sin(q1R))/20282409603651670423947251286016 + 2903273033334964234439083875867/41538374868278621028243970633760768))/81129638414606681695789005144064 - (14115856197532180673579726082375*sin(q2R)*((1392340654334763*cos(q1R))/2251799813685248 + (398031123528767*sin(q1R))/562949953421312))/340282366920938463463374607431768211456 + (2115063383689692319117831580025*sin(q3R)*((3585145564851136108341178694895*cos(q1R))/5070602400912917605986812821504 - (12541089443950065443620820128155*sin(q1R))/20282409603651670423947251286016 + 2903273033334964234439083875867/41538374868278621028243970633760768))/10384593717069655257060992658440192 + 34189201462609793352471527538206775118278208232606556159508725/57896044618658097711785492504343953926634992332820282019728792003956564819968))/119726214130147567059245861496117904970213993920593920, (202883803014822867*cos(q6R)*((7514214926474921*cos(q5R)*(((4503599440548691*cos(q4R))/4503599627370496 - (7514214926474921*sin(q4R))/36893488147419103232)*(cos(q3R)*((3480118470877607344838997022995*sin(q2R))/10141204801825835211973625643008 + cos(q2R)*((1392340654334763*cos(q1R))/2251799813685248 + (398031123528767*sin(q1R))/562949953421312) - (7514214926474921*sin(q2R)*((398031123528767*cos(q1R))/562949953421312 - (1392340654334763*sin(q1R))/2251799813685248))/36893488147419103232) + (7514214926474921*sin(q3R)*((7514214926474921*cos(q2R)*((398031123528767*cos(q1R))/562949953421312 - (1392340654334763*sin(q1R))/2251799813685248))/36893488147419103232 - (3480118470877607344838997022995*cos(q2R))/10141204801825835211973625643008 + sin(q2R)*((1392340654334763*cos(q1R))/2251799813685248 + (398031123528767*sin(q1R))/562949953421312)))/36893488147419103232 + (9007199067919185*sin(q3R)*((3585145564851136108341178694895*cos(q1R))/5070602400912917605986812821504 - (12541089443950065443620820128155*sin(q1R))/20282409603651670423947251286016 + 2903273033334964234439083875867/41538374868278621028243970633760768))/9007199254740992) + ((234819211581865*cos(q4R))/1152921504606846976 + (9007199067919185*sin(q4R))/9007199254740992)*((26939554316989768830159504461322709929728228295*cos(q1R))/187072209578355573530071658587684226515959365500928 + (31346119847137124244279794758002175024246659075*cos(q2R))/91343852333181432387730302044767688728495783936 - (94236441493986648894942587121893377357613500755*sin(q1R))/748288838313422294120286634350736906063837462003712 - (67682029681889335677290557259385*cos(q2R)*((398031123528767*cos(q1R))/562949953421312 - (1392340654334763*sin(q1R))/2251799813685248))/332306998946228968225951765070086144 - (9007199067919185*sin(q2R)*((1392340654334763*cos(q1R))/2251799813685248 + (398031123528767*sin(q1R))/562949953421312))/9007199254740992 + 21815817562717709140362801846989786744252631507/1532495540865888858358347027150309183618739122183602176) + (7514214926474921*cos(q4R)*((7514214926474921*cos(q3R)*((7514214926474921*cos(q2R)*((398031123528767*cos(q1R))/562949953421312 - (1392340654334763*sin(q1R))/2251799813685248))/36893488147419103232 - (3480118470877607344838997022995*cos(q2R))/10141204801825835211973625643008 + sin(q2R)*((1392340654334763*cos(q1R))/2251799813685248 + (398031123528767*sin(q1R))/562949953421312)))/36893488147419103232 - sin(q3R)*((3480118470877607344838997022995*sin(q2R))/10141204801825835211973625643008 + cos(q2R)*((1392340654334763*cos(q1R))/2251799813685248 + (398031123528767*sin(q1R))/562949953421312) - (7514214926474921*sin(q2R)*((398031123528767*cos(q1R))/562949953421312 - (1392340654334763*sin(q1R))/2251799813685248))/36893488147419103232) + (9007199067919185*cos(q3R)*((3585145564851136108341178694895*cos(q1R))/5070602400912917605986812821504 - (12541089443950065443620820128155*sin(q1R))/20282409603651670423947251286016 + 2903273033334964234439083875867/41538374868278621028243970633760768))/9007199254740992))/36893488147419103232))/36893488147419103232 + sin(q5R)*((7514214926474921*sin(q4R)*((7514214926474921*cos(q3R)*((7514214926474921*cos(q2R)*((398031123528767*cos(q1R))/562949953421312 - (1392340654334763*sin(q1R))/2251799813685248))/36893488147419103232 - (3480118470877607344838997022995*cos(q2R))/10141204801825835211973625643008 + sin(q2R)*((1392340654334763*cos(q1R))/2251799813685248 + (398031123528767*sin(q1R))/562949953421312)))/36893488147419103232 - sin(q3R)*((3480118470877607344838997022995*sin(q2R))/10141204801825835211973625643008 + cos(q2R)*((1392340654334763*cos(q1R))/2251799813685248 + (398031123528767*sin(q1R))/562949953421312) - (7514214926474921*sin(q2R)*((398031123528767*cos(q1R))/562949953421312 - (1392340654334763*sin(q1R))/2251799813685248))/36893488147419103232) + (9007199067919185*cos(q3R)*((3585145564851136108341178694895*cos(q1R))/5070602400912917605986812821504 - (12541089443950065443620820128155*sin(q1R))/20282409603651670423947251286016 + 2903273033334964234439083875867/41538374868278621028243970633760768))/9007199254740992))/36893488147419103232 + ((7514214926474921*cos(q4R))/36893488147419103232 + (4503599440548691*sin(q4R))/4503599627370496)*(cos(q3R)*((3480118470877607344838997022995*sin(q2R))/10141204801825835211973625643008 + cos(q2R)*((1392340654334763*cos(q1R))/2251799813685248 + (398031123528767*sin(q1R))/562949953421312) - (7514214926474921*sin(q2R)*((398031123528767*cos(q1R))/562949953421312 - (1392340654334763*sin(q1R))/2251799813685248))/36893488147419103232) + (7514214926474921*sin(q3R)*((7514214926474921*cos(q2R)*((398031123528767*cos(q1R))/562949953421312 - (1392340654334763*sin(q1R))/2251799813685248))/36893488147419103232 - (3480118470877607344838997022995*cos(q2R))/10141204801825835211973625643008 + sin(q2R)*((1392340654334763*cos(q1R))/2251799813685248 + (398031123528767*sin(q1R))/562949953421312)))/36893488147419103232 + (9007199067919185*sin(q3R)*((3585145564851136108341178694895*cos(q1R))/5070602400912917605986812821504 - (12541089443950065443620820128155*sin(q1R))/20282409603651670423947251286016 + 2903273033334964234439083875867/41538374868278621028243970633760768))/9007199254740992) - ((9007199067919185*cos(q4R))/9007199254740992 - (234819211581865*sin(q4R))/1152921504606846976)*((26939554316989768830159504461322709929728228295*cos(q1R))/187072209578355573530071658587684226515959365500928 + (31346119847137124244279794758002175024246659075*cos(q2R))/91343852333181432387730302044767688728495783936 - (94236441493986648894942587121893377357613500755*sin(q1R))/748288838313422294120286634350736906063837462003712 - (67682029681889335677290557259385*cos(q2R)*((398031123528767*cos(q1R))/562949953421312 - (1392340654334763*sin(q1R))/2251799813685248))/332306998946228968225951765070086144 - (9007199067919185*sin(q2R)*((1392340654334763*cos(q1R))/2251799813685248 + (398031123528767*sin(q1R))/562949953421312))/9007199254740992 + 21815817562717709140362801846989786744252631507/1532495540865888858358347027150309183618739122183602176)) - (9007199067919185*cos(q5R)*((42218993040650622024393554167529407181397382817729417611526625*cos(q1R))/7067388259113537318333190002971674063309935587502475832486424805170479104 + (49124851885283889459147163519037433596494512994900179139213125*cos(q2R))/3450873173395281893717377931138512726225554486085193277581262111899648 - (147684984717849177105467939785270041851792306559769220895307125*sin(q1R))/28269553036454149273332760011886696253239742350009903329945699220681916416 - (67682029681889335677290557259385*cos(q3R)*((7514214926474921*cos(q2R)*((398031123528767*cos(q1R))/562949953421312 - (1392340654334763*sin(q1R))/2251799813685248))/36893488147419103232 - (3480118470877607344838997022995*cos(q2R))/10141204801825835211973625643008 + sin(q2R)*((1392340654334763*cos(q1R))/2251799813685248 + (398031123528767*sin(q1R))/562949953421312)))/332306998946228968225951765070086144 + (234819211581865*cos(q3R)*((3480118470877607344838997022995*sin(q2R))/10141204801825835211973625643008 + cos(q2R)*((1392340654334763*cos(q1R))/2251799813685248 + (398031123528767*sin(q1R))/562949953421312) - (7514214926474921*sin(q2R)*((398031123528767*cos(q1R))/562949953421312 - (1392340654334763*sin(q1R))/2251799813685248))/36893488147419103232))/1152921504606846976 + (1764482024691522628700660907665*sin(q3R)*((7514214926474921*cos(q2R)*((398031123528767*cos(q1R))/562949953421312 - (1392340654334763*sin(q1R))/2251799813685248))/36893488147419103232 - (3480118470877607344838997022995*cos(q2R))/10141204801825835211973625643008 + sin(q2R)*((1392340654334763*cos(q1R))/2251799813685248 + (398031123528767*sin(q1R))/562949953421312)))/42535295865117307932921825928971026432 + (9007199067919185*sin(q3R)*((3480118470877607344838997022995*sin(q2R))/10141204801825835211973625643008 + cos(q2R)*((1392340654334763*cos(q1R))/2251799813685248 + (398031123528767*sin(q1R))/562949953421312) - (7514214926474921*sin(q2R)*((398031123528767*cos(q1R))/562949953421312 - (1392340654334763*sin(q1R))/2251799813685248))/36893488147419103232))/9007199254740992 - (106069577339469832923929692356850887620017617375*cos(q2R)*((398031123528767*cos(q1R))/562949953421312 - (1392340654334763*sin(q1R))/2251799813685248))/12554203470773361527671578846415332832204710888928069025792 - (81129635049124235038645691064225*cos(q3R)*((3585145564851136108341178694895*cos(q1R))/5070602400912917605986812821504 - (12541089443950065443620820128155*sin(q1R))/20282409603651670423947251286016 + 2903273033334964234439083875867/41538374868278621028243970633760768))/81129638414606681695789005144064 - (14115856197532180673579726082375*sin(q2R)*((1392340654334763*cos(q1R))/2251799813685248 + (398031123528767*sin(q1R))/562949953421312))/340282366920938463463374607431768211456 + (2115063383689692319117831580025*sin(q3R)*((3585145564851136108341178694895*cos(q1R))/5070602400912917605986812821504 - (12541089443950065443620820128155*sin(q1R))/20282409603651670423947251286016 + 2903273033334964234439083875867/41538374868278621028243970633760768))/10384593717069655257060992658440192 + 34189201462609793352471527538206775118278208232606556159508725/57896044618658097711785492504343953926634992332820282019728792003956564819968))/9007199254740992))/36893488147419103232000 - (584133382113593486367040631332731*sin(q6R)*((317242587686797715160741214886285987125185037094314753690999507962888586271625*cos(q1R))/260740604970814219042361048116400404614587954389239840081425977517360806369707098391474864128 + (369134695297269865703468593411141398729137707824460658574000083747077986538125*cos(q2R))/127314748520905380391777855525586135065716774604121015664758778084648831235208544136462336 - (1109736716583082885849910318389051322854142663349680644790580040185967905112125*sin(q1R))/1042962419883256876169444192465601618458351817556959360325703910069443225478828393565899456512 - (508577317689771495245073589786522929324694383585*cos(q3R)*((7514214926474921*cos(q2R)*((398031123528767*cos(q1R))/562949953421312 - (1392340654334763*sin(q1R))/2251799813685248))/36893488147419103232 - (3480118470877607344838997022995*cos(q2R))/10141204801825835211973625643008 + sin(q2R)*((1392340654334763*cos(q1R))/2251799813685248 + (398031123528767*sin(q1R))/562949953421312)))/12259964326927110866866776217202473468949912977468817408 + (1764482024691522628700660907665*cos(q3R)*((3480118470877607344838997022995*sin(q2R))/10141204801825835211973625643008 + cos(q2R)*((1392340654334763*cos(q1R))/2251799813685248 + (398031123528767*sin(q1R))/562949953421312) - (7514214926474921*sin(q2R)*((398031123528767*cos(q1R))/562949953421312 - (1392340654334763*sin(q1R))/2251799813685248))/36893488147419103232))/42535295865117307932921825928971026432 + (13258697167433729449897784796786197386719169465*sin(q3R)*((7514214926474921*cos(q2R)*((398031123528767*cos(q1R))/562949953421312 - (1392340654334763*sin(q1R))/2251799813685248))/36893488147419103232 - (3480118470877607344838997022995*cos(q2R))/10141204801825835211973625643008 + sin(q2R)*((1392340654334763*cos(q1R))/2251799813685248 + (398031123528767*sin(q1R))/562949953421312)))/1569275433846670190958947355801916604025588861116008628224 + (67682029681889335677290557259385*sin(q3R)*((3480118470877607344838997022995*sin(q2R))/10141204801825835211973625643008 + cos(q2R)*((1392340654334763*cos(q1R))/2251799813685248 + (398031123528767*sin(q1R))/562949953421312) - (7514214926474921*sin(q2R)*((398031123528767*cos(q1R))/562949953421312 - (1392340654334763*sin(q1R))/2251799813685248))/36893488147419103232))/332306998946228968225951765070086144 - (797029601289130257223357069404502671534492977261568326111352375*cos(q2R)*((398031123528767*cos(q1R))/562949953421312 - (1392340654334763*sin(q1R))/2251799813685248))/463168356949264781694283940034751631413079938662562256157830336031652518559744 - (609625514665592237562888769449172969868262801225*cos(q3R)*((3585145564851136108341178694895*cos(q1R))/5070602400912917605986812821504 - (12541089443950065443620820128155*sin(q1R))/20282409603651670423947251286016 + 2903273033334964234439083875867/41538374868278621028243970633760768))/2993155353253689176481146537402947624255349848014848 + (9007199067919185*((4503599440548691*cos(q4R))/4503599627370496 - (7514214926474921*sin(q4R))/36893488147419103232)*(cos(q3R)*((3480118470877607344838997022995*sin(q2R))/10141204801825835211973625643008 + cos(q2R)*((1392340654334763*cos(q1R))/2251799813685248 + (398031123528767*sin(q1R))/562949953421312) - (7514214926474921*sin(q2R)*((398031123528767*cos(q1R))/562949953421312 - (1392340654334763*sin(q1R))/2251799813685248))/36893488147419103232) + (7514214926474921*sin(q3R)*((7514214926474921*cos(q2R)*((398031123528767*cos(q1R))/562949953421312 - (1392340654334763*sin(q1R))/2251799813685248))/36893488147419103232 - (3480118470877607344838997022995*cos(q2R))/10141204801825835211973625643008 + sin(q2R)*((1392340654334763*cos(q1R))/2251799813685248 + (398031123528767*sin(q1R))/562949953421312)))/36893488147419103232 + (9007199067919185*sin(q3R)*((3585145564851136108341178694895*cos(q1R))/5070602400912917605986812821504 - (12541089443950065443620820128155*sin(q1R))/20282409603651670423947251286016 + 2903273033334964234439083875867/41538374868278621028243970633760768))/9007199254740992))/9007199254740992 - (106069577339469832923929692356850887620017617375*sin(q2R)*((1392340654334763*cos(q1R))/2251799813685248 + (398031123528767*sin(q1R))/562949953421312))/12554203470773361527671578846415332832204710888928069025792 + (15893040848161638993908057577265778144967053025*sin(q3R)*((3585145564851136108341178694895*cos(q1R))/5070602400912917605986812821504 - (12541089443950065443620820128155*sin(q1R))/20282409603651670423947251286016 + 2903273033334964234439083875867/41538374868278621028243970633760768))/383123885216472214589586756787577295904684780545900544 + (9007199067919185*((234819211581865*cos(q4R))/1152921504606846976 + (9007199067919185*sin(q4R))/9007199254740992)*((26939554316989768830159504461322709929728228295*cos(q1R))/187072209578355573530071658587684226515959365500928 + (31346119847137124244279794758002175024246659075*cos(q2R))/91343852333181432387730302044767688728495783936 - (94236441493986648894942587121893377357613500755*sin(q1R))/748288838313422294120286634350736906063837462003712 - (67682029681889335677290557259385*cos(q2R)*((398031123528767*cos(q1R))/562949953421312 - (1392340654334763*sin(q1R))/2251799813685248))/332306998946228968225951765070086144 - (9007199067919185*sin(q2R)*((1392340654334763*cos(q1R))/2251799813685248 + (398031123528767*sin(q1R))/562949953421312))/9007199254740992 + 21815817562717709140362801846989786744252631507/1532495540865888858358347027150309183618739122183602176))/9007199254740992 + (67682029681889335677290557259385*cos(q4R)*((7514214926474921*cos(q3R)*((7514214926474921*cos(q2R)*((398031123528767*cos(q1R))/562949953421312 - (1392340654334763*sin(q1R))/2251799813685248))/36893488147419103232 - (3480118470877607344838997022995*cos(q2R))/10141204801825835211973625643008 + sin(q2R)*((1392340654334763*cos(q1R))/2251799813685248 + (398031123528767*sin(q1R))/562949953421312)))/36893488147419103232 - sin(q3R)*((3480118470877607344838997022995*sin(q2R))/10141204801825835211973625643008 + cos(q2R)*((1392340654334763*cos(q1R))/2251799813685248 + (398031123528767*sin(q1R))/562949953421312) - (7514214926474921*sin(q2R)*((398031123528767*cos(q1R))/562949953421312 - (1392340654334763*sin(q1R))/2251799813685248))/36893488147419103232) + (9007199067919185*cos(q3R)*((3585145564851136108341178694895*cos(q1R))/5070602400912917605986812821504 - (12541089443950065443620820128155*sin(q1R))/20282409603651670423947251286016 + 2903273033334964234439083875867/41538374868278621028243970633760768))/9007199254740992))/332306998946228968225951765070086144 + 256905007954600709870741236886362515198064227567936069111275436480059393185725/2135987035920910082395021706169552114602704522356652769947041607822219725780640550022962086936576))/16225927682921336339157801028812800 - (324259171862923063*cos(q6R)*(cos(q5R)*((7514214926474921*sin(q4R)*((7514214926474921*cos(q3R)*((7514214926474921*cos(q2R)*((398031123528767*cos(q1R))/562949953421312 - (1392340654334763*sin(q1R))/2251799813685248))/36893488147419103232 - (3480118470877607344838997022995*cos(q2R))/10141204801825835211973625643008 + sin(q2R)*((1392340654334763*cos(q1R))/2251799813685248 + (398031123528767*sin(q1R))/562949953421312)))/36893488147419103232 - sin(q3R)*((3480118470877607344838997022995*sin(q2R))/10141204801825835211973625643008 + cos(q2R)*((1392340654334763*cos(q1R))/2251799813685248 + (398031123528767*sin(q1R))/562949953421312) - (7514214926474921*sin(q2R)*((398031123528767*cos(q1R))/562949953421312 - (1392340654334763*sin(q1R))/2251799813685248))/36893488147419103232) + (9007199067919185*cos(q3R)*((3585145564851136108341178694895*cos(q1R))/5070602400912917605986812821504 - (12541089443950065443620820128155*sin(q1R))/20282409603651670423947251286016 + 2903273033334964234439083875867/41538374868278621028243970633760768))/9007199254740992))/36893488147419103232 + ((7514214926474921*cos(q4R))/36893488147419103232 + (4503599440548691*sin(q4R))/4503599627370496)*(cos(q3R)*((3480118470877607344838997022995*sin(q2R))/10141204801825835211973625643008 + cos(q2R)*((1392340654334763*cos(q1R))/2251799813685248 + (398031123528767*sin(q1R))/562949953421312) - (7514214926474921*sin(q2R)*((398031123528767*cos(q1R))/562949953421312 - (1392340654334763*sin(q1R))/2251799813685248))/36893488147419103232) + (7514214926474921*sin(q3R)*((7514214926474921*cos(q2R)*((398031123528767*cos(q1R))/562949953421312 - (1392340654334763*sin(q1R))/2251799813685248))/36893488147419103232 - (3480118470877607344838997022995*cos(q2R))/10141204801825835211973625643008 + sin(q2R)*((1392340654334763*cos(q1R))/2251799813685248 + (398031123528767*sin(q1R))/562949953421312)))/36893488147419103232 + (9007199067919185*sin(q3R)*((3585145564851136108341178694895*cos(q1R))/5070602400912917605986812821504 - (12541089443950065443620820128155*sin(q1R))/20282409603651670423947251286016 + 2903273033334964234439083875867/41538374868278621028243970633760768))/9007199254740992) - ((9007199067919185*cos(q4R))/9007199254740992 - (234819211581865*sin(q4R))/1152921504606846976)*((26939554316989768830159504461322709929728228295*cos(q1R))/187072209578355573530071658587684226515959365500928 + (31346119847137124244279794758002175024246659075*cos(q2R))/91343852333181432387730302044767688728495783936 - (94236441493986648894942587121893377357613500755*sin(q1R))/748288838313422294120286634350736906063837462003712 - (67682029681889335677290557259385*cos(q2R)*((398031123528767*cos(q1R))/562949953421312 - (1392340654334763*sin(q1R))/2251799813685248))/332306998946228968225951765070086144 - (9007199067919185*sin(q2R)*((1392340654334763*cos(q1R))/2251799813685248 + (398031123528767*sin(q1R))/562949953421312))/9007199254740992 + 21815817562717709140362801846989786744252631507/1532495540865888858358347027150309183618739122183602176)) - (7514214926474921*sin(q5R)*(((4503599440548691*cos(q4R))/4503599627370496 - (7514214926474921*sin(q4R))/36893488147419103232)*(cos(q3R)*((3480118470877607344838997022995*sin(q2R))/10141204801825835211973625643008 + cos(q2R)*((1392340654334763*cos(q1R))/2251799813685248 + (398031123528767*sin(q1R))/562949953421312) - (7514214926474921*sin(q2R)*((398031123528767*cos(q1R))/562949953421312 - (1392340654334763*sin(q1R))/2251799813685248))/36893488147419103232) + (7514214926474921*sin(q3R)*((7514214926474921*cos(q2R)*((398031123528767*cos(q1R))/562949953421312 - (1392340654334763*sin(q1R))/2251799813685248))/36893488147419103232 - (3480118470877607344838997022995*cos(q2R))/10141204801825835211973625643008 + sin(q2R)*((1392340654334763*cos(q1R))/2251799813685248 + (398031123528767*sin(q1R))/562949953421312)))/36893488147419103232 + (9007199067919185*sin(q3R)*((3585145564851136108341178694895*cos(q1R))/5070602400912917605986812821504 - (12541089443950065443620820128155*sin(q1R))/20282409603651670423947251286016 + 2903273033334964234439083875867/41538374868278621028243970633760768))/9007199254740992) + ((234819211581865*cos(q4R))/1152921504606846976 + (9007199067919185*sin(q4R))/9007199254740992)*((26939554316989768830159504461322709929728228295*cos(q1R))/187072209578355573530071658587684226515959365500928 + (31346119847137124244279794758002175024246659075*cos(q2R))/91343852333181432387730302044767688728495783936 - (94236441493986648894942587121893377357613500755*sin(q1R))/748288838313422294120286634350736906063837462003712 - (67682029681889335677290557259385*cos(q2R)*((398031123528767*cos(q1R))/562949953421312 - (1392340654334763*sin(q1R))/2251799813685248))/332306998946228968225951765070086144 - (9007199067919185*sin(q2R)*((1392340654334763*cos(q1R))/2251799813685248 + (398031123528767*sin(q1R))/562949953421312))/9007199254740992 + 21815817562717709140362801846989786744252631507/1532495540865888858358347027150309183618739122183602176) + (7514214926474921*cos(q4R)*((7514214926474921*cos(q3R)*((7514214926474921*cos(q2R)*((398031123528767*cos(q1R))/562949953421312 - (1392340654334763*sin(q1R))/2251799813685248))/36893488147419103232 - (3480118470877607344838997022995*cos(q2R))/10141204801825835211973625643008 + sin(q2R)*((1392340654334763*cos(q1R))/2251799813685248 + (398031123528767*sin(q1R))/562949953421312)))/36893488147419103232 - sin(q3R)*((3480118470877607344838997022995*sin(q2R))/10141204801825835211973625643008 + cos(q2R)*((1392340654334763*cos(q1R))/2251799813685248 + (398031123528767*sin(q1R))/562949953421312) - (7514214926474921*sin(q2R)*((398031123528767*cos(q1R))/562949953421312 - (1392340654334763*sin(q1R))/2251799813685248))/36893488147419103232) + (9007199067919185*cos(q3R)*((3585145564851136108341178694895*cos(q1R))/5070602400912917605986812821504 - (12541089443950065443620820128155*sin(q1R))/20282409603651670423947251286016 + 2903273033334964234439083875867/41538374868278621028243970633760768))/9007199254740992))/36893488147419103232))/36893488147419103232 + (9007199067919185*sin(q5R)*((42218993040650622024393554167529407181397382817729417611526625*cos(q1R))/7067388259113537318333190002971674063309935587502475832486424805170479104 + (49124851885283889459147163519037433596494512994900179139213125*cos(q2R))/3450873173395281893717377931138512726225554486085193277581262111899648 - (147684984717849177105467939785270041851792306559769220895307125*sin(q1R))/28269553036454149273332760011886696253239742350009903329945699220681916416 - (67682029681889335677290557259385*cos(q3R)*((7514214926474921*cos(q2R)*((398031123528767*cos(q1R))/562949953421312 - (1392340654334763*sin(q1R))/2251799813685248))/36893488147419103232 - (3480118470877607344838997022995*cos(q2R))/10141204801825835211973625643008 + sin(q2R)*((1392340654334763*cos(q1R))/2251799813685248 + (398031123528767*sin(q1R))/562949953421312)))/332306998946228968225951765070086144 + (234819211581865*cos(q3R)*((3480118470877607344838997022995*sin(q2R))/10141204801825835211973625643008 + cos(q2R)*((1392340654334763*cos(q1R))/2251799813685248 + (398031123528767*sin(q1R))/562949953421312) - (7514214926474921*sin(q2R)*((398031123528767*cos(q1R))/562949953421312 - (1392340654334763*sin(q1R))/2251799813685248))/36893488147419103232))/1152921504606846976 + (1764482024691522628700660907665*sin(q3R)*((7514214926474921*cos(q2R)*((398031123528767*cos(q1R))/562949953421312 - (1392340654334763*sin(q1R))/2251799813685248))/36893488147419103232 - (3480118470877607344838997022995*cos(q2R))/10141204801825835211973625643008 + sin(q2R)*((1392340654334763*cos(q1R))/2251799813685248 + (398031123528767*sin(q1R))/562949953421312)))/42535295865117307932921825928971026432 + (9007199067919185*sin(q3R)*((3480118470877607344838997022995*sin(q2R))/10141204801825835211973625643008 + cos(q2R)*((1392340654334763*cos(q1R))/2251799813685248 + (398031123528767*sin(q1R))/562949953421312) - (7514214926474921*sin(q2R)*((398031123528767*cos(q1R))/562949953421312 - (1392340654334763*sin(q1R))/2251799813685248))/36893488147419103232))/9007199254740992 - (106069577339469832923929692356850887620017617375*cos(q2R)*((398031123528767*cos(q1R))/562949953421312 - (1392340654334763*sin(q1R))/2251799813685248))/12554203470773361527671578846415332832204710888928069025792 - (81129635049124235038645691064225*cos(q3R)*((3585145564851136108341178694895*cos(q1R))/5070602400912917605986812821504 - (12541089443950065443620820128155*sin(q1R))/20282409603651670423947251286016 + 2903273033334964234439083875867/41538374868278621028243970633760768))/81129638414606681695789005144064 - (14115856197532180673579726082375*sin(q2R)*((1392340654334763*cos(q1R))/2251799813685248 + (398031123528767*sin(q1R))/562949953421312))/340282366920938463463374607431768211456 + (2115063383689692319117831580025*sin(q3R)*((3585145564851136108341178694895*cos(q1R))/5070602400912917605986812821504 - (12541089443950065443620820128155*sin(q1R))/20282409603651670423947251286016 + 2903273033334964234439083875867/41538374868278621028243970633760768))/10384593717069655257060992658440192 + 34189201462609793352471527538206775118278208232606556159508725/57896044618658097711785492504343953926634992332820282019728792003956564819968))/9007199254740992))/9007199254740992000 - (2436553109258773196144549622003023*sin(q6R)*((7514214926474921*cos(q5R)*(((4503599440548691*cos(q4R))/4503599627370496 - (7514214926474921*sin(q4R))/36893488147419103232)*(cos(q3R)*((3480118470877607344838997022995*sin(q2R))/10141204801825835211973625643008 + cos(q2R)*((1392340654334763*cos(q1R))/2251799813685248 + (398031123528767*sin(q1R))/562949953421312) - (7514214926474921*sin(q2R)*((398031123528767*cos(q1R))/562949953421312 - (1392340654334763*sin(q1R))/2251799813685248))/36893488147419103232) + (7514214926474921*sin(q3R)*((7514214926474921*cos(q2R)*((398031123528767*cos(q1R))/562949953421312 - (1392340654334763*sin(q1R))/2251799813685248))/36893488147419103232 - (3480118470877607344838997022995*cos(q2R))/10141204801825835211973625643008 + sin(q2R)*((1392340654334763*cos(q1R))/2251799813685248 + (398031123528767*sin(q1R))/562949953421312)))/36893488147419103232 + (9007199067919185*sin(q3R)*((3585145564851136108341178694895*cos(q1R))/5070602400912917605986812821504 - (12541089443950065443620820128155*sin(q1R))/20282409603651670423947251286016 + 2903273033334964234439083875867/41538374868278621028243970633760768))/9007199254740992) + ((234819211581865*cos(q4R))/1152921504606846976 + (9007199067919185*sin(q4R))/9007199254740992)*((26939554316989768830159504461322709929728228295*cos(q1R))/187072209578355573530071658587684226515959365500928 + (31346119847137124244279794758002175024246659075*cos(q2R))/91343852333181432387730302044767688728495783936 - (94236441493986648894942587121893377357613500755*sin(q1R))/748288838313422294120286634350736906063837462003712 - (67682029681889335677290557259385*cos(q2R)*((398031123528767*cos(q1R))/562949953421312 - (1392340654334763*sin(q1R))/2251799813685248))/332306998946228968225951765070086144 - (9007199067919185*sin(q2R)*((1392340654334763*cos(q1R))/2251799813685248 + (398031123528767*sin(q1R))/562949953421312))/9007199254740992 + 21815817562717709140362801846989786744252631507/1532495540865888858358347027150309183618739122183602176) + (7514214926474921*cos(q4R)*((7514214926474921*cos(q3R)*((7514214926474921*cos(q2R)*((398031123528767*cos(q1R))/562949953421312 - (1392340654334763*sin(q1R))/2251799813685248))/36893488147419103232 - (3480118470877607344838997022995*cos(q2R))/10141204801825835211973625643008 + sin(q2R)*((1392340654334763*cos(q1R))/2251799813685248 + (398031123528767*sin(q1R))/562949953421312)))/36893488147419103232 - sin(q3R)*((3480118470877607344838997022995*sin(q2R))/10141204801825835211973625643008 + cos(q2R)*((1392340654334763*cos(q1R))/2251799813685248 + (398031123528767*sin(q1R))/562949953421312) - (7514214926474921*sin(q2R)*((398031123528767*cos(q1R))/562949953421312 - (1392340654334763*sin(q1R))/2251799813685248))/36893488147419103232) + (9007199067919185*cos(q3R)*((3585145564851136108341178694895*cos(q1R))/5070602400912917605986812821504 - (12541089443950065443620820128155*sin(q1R))/20282409603651670423947251286016 + 2903273033334964234439083875867/41538374868278621028243970633760768))/9007199254740992))/36893488147419103232))/36893488147419103232 + sin(q5R)*((7514214926474921*sin(q4R)*((7514214926474921*cos(q3R)*((7514214926474921*cos(q2R)*((398031123528767*cos(q1R))/562949953421312 - (1392340654334763*sin(q1R))/2251799813685248))/36893488147419103232 - (3480118470877607344838997022995*cos(q2R))/10141204801825835211973625643008 + sin(q2R)*((1392340654334763*cos(q1R))/2251799813685248 + (398031123528767*sin(q1R))/562949953421312)))/36893488147419103232 - sin(q3R)*((3480118470877607344838997022995*sin(q2R))/10141204801825835211973625643008 + cos(q2R)*((1392340654334763*cos(q1R))/2251799813685248 + (398031123528767*sin(q1R))/562949953421312) - (7514214926474921*sin(q2R)*((398031123528767*cos(q1R))/562949953421312 - (1392340654334763*sin(q1R))/2251799813685248))/36893488147419103232) + (9007199067919185*cos(q3R)*((3585145564851136108341178694895*cos(q1R))/5070602400912917605986812821504 - (12541089443950065443620820128155*sin(q1R))/20282409603651670423947251286016 + 2903273033334964234439083875867/41538374868278621028243970633760768))/9007199254740992))/36893488147419103232 + ((7514214926474921*cos(q4R))/36893488147419103232 + (4503599440548691*sin(q4R))/4503599627370496)*(cos(q3R)*((3480118470877607344838997022995*sin(q2R))/10141204801825835211973625643008 + cos(q2R)*((1392340654334763*cos(q1R))/2251799813685248 + (398031123528767*sin(q1R))/562949953421312) - (7514214926474921*sin(q2R)*((398031123528767*cos(q1R))/562949953421312 - (1392340654334763*sin(q1R))/2251799813685248))/36893488147419103232) + (7514214926474921*sin(q3R)*((7514214926474921*cos(q2R)*((398031123528767*cos(q1R))/562949953421312 - (1392340654334763*sin(q1R))/2251799813685248))/36893488147419103232 - (3480118470877607344838997022995*cos(q2R))/10141204801825835211973625643008 + sin(q2R)*((1392340654334763*cos(q1R))/2251799813685248 + (398031123528767*sin(q1R))/562949953421312)))/36893488147419103232 + (9007199067919185*sin(q3R)*((3585145564851136108341178694895*cos(q1R))/5070602400912917605986812821504 - (12541089443950065443620820128155*sin(q1R))/20282409603651670423947251286016 + 2903273033334964234439083875867/41538374868278621028243970633760768))/9007199254740992) - ((9007199067919185*cos(q4R))/9007199254740992 - (234819211581865*sin(q4R))/1152921504606846976)*((26939554316989768830159504461322709929728228295*cos(q1R))/187072209578355573530071658587684226515959365500928 + (31346119847137124244279794758002175024246659075*cos(q2R))/91343852333181432387730302044767688728495783936 - (94236441493986648894942587121893377357613500755*sin(q1R))/748288838313422294120286634350736906063837462003712 - (67682029681889335677290557259385*cos(q2R)*((398031123528767*cos(q1R))/562949953421312 - (1392340654334763*sin(q1R))/2251799813685248))/332306998946228968225951765070086144 - (9007199067919185*sin(q2R)*((1392340654334763*cos(q1R))/2251799813685248 + (398031123528767*sin(q1R))/562949953421312))/9007199254740992 + 21815817562717709140362801846989786744252631507/1532495540865888858358347027150309183618739122183602176)) - (9007199067919185*cos(q5R)*((42218993040650622024393554167529407181397382817729417611526625*cos(q1R))/7067388259113537318333190002971674063309935587502475832486424805170479104 + (49124851885283889459147163519037433596494512994900179139213125*cos(q2R))/3450873173395281893717377931138512726225554486085193277581262111899648 - (147684984717849177105467939785270041851792306559769220895307125*sin(q1R))/28269553036454149273332760011886696253239742350009903329945699220681916416 - (67682029681889335677290557259385*cos(q3R)*((7514214926474921*cos(q2R)*((398031123528767*cos(q1R))/562949953421312 - (1392340654334763*sin(q1R))/2251799813685248))/36893488147419103232 - (3480118470877607344838997022995*cos(q2R))/10141204801825835211973625643008 + sin(q2R)*((1392340654334763*cos(q1R))/2251799813685248 + (398031123528767*sin(q1R))/562949953421312)))/332306998946228968225951765070086144 + (234819211581865*cos(q3R)*((3480118470877607344838997022995*sin(q2R))/10141204801825835211973625643008 + cos(q2R)*((1392340654334763*cos(q1R))/2251799813685248 + (398031123528767*sin(q1R))/562949953421312) - (7514214926474921*sin(q2R)*((398031123528767*cos(q1R))/562949953421312 - (1392340654334763*sin(q1R))/2251799813685248))/36893488147419103232))/1152921504606846976 + (1764482024691522628700660907665*sin(q3R)*((7514214926474921*cos(q2R)*((398031123528767*cos(q1R))/562949953421312 - (1392340654334763*sin(q1R))/2251799813685248))/36893488147419103232 - (3480118470877607344838997022995*cos(q2R))/10141204801825835211973625643008 + sin(q2R)*((1392340654334763*cos(q1R))/2251799813685248 + (398031123528767*sin(q1R))/562949953421312)))/42535295865117307932921825928971026432 + (9007199067919185*sin(q3R)*((3480118470877607344838997022995*sin(q2R))/10141204801825835211973625643008 + cos(q2R)*((1392340654334763*cos(q1R))/2251799813685248 + (398031123528767*sin(q1R))/562949953421312) - (7514214926474921*sin(q2R)*((398031123528767*cos(q1R))/562949953421312 - (1392340654334763*sin(q1R))/2251799813685248))/36893488147419103232))/9007199254740992 - (106069577339469832923929692356850887620017617375*cos(q2R)*((398031123528767*cos(q1R))/562949953421312 - (1392340654334763*sin(q1R))/2251799813685248))/12554203470773361527671578846415332832204710888928069025792 - (81129635049124235038645691064225*cos(q3R)*((3585145564851136108341178694895*cos(q1R))/5070602400912917605986812821504 - (12541089443950065443620820128155*sin(q1R))/20282409603651670423947251286016 + 2903273033334964234439083875867/41538374868278621028243970633760768))/81129638414606681695789005144064 - (14115856197532180673579726082375*sin(q2R)*((1392340654334763*cos(q1R))/2251799813685248 + (398031123528767*sin(q1R))/562949953421312))/340282366920938463463374607431768211456 + (2115063383689692319117831580025*sin(q3R)*((3585145564851136108341178694895*cos(q1R))/5070602400912917605986812821504 - (12541089443950065443620820128155*sin(q1R))/20282409603651670423947251286016 + 2903273033334964234439083875867/41538374868278621028243970633760768))/10384593717069655257060992658440192 + 34189201462609793352471527538206775118278208232606556159508725/57896044618658097711785492504343953926634992332820282019728792003956564819968))/9007199254740992))/332306998946228968225951765070086144000 - (27*sin(q6R)*(cos(q5R)*((7514214926474921*sin(q4R)*((7514214926474921*cos(q3R)*((7514214926474921*cos(q2R)*((398031123528767*cos(q1R))/562949953421312 - (1392340654334763*sin(q1R))/2251799813685248))/36893488147419103232 - (3480118470877607344838997022995*cos(q2R))/10141204801825835211973625643008 + sin(q2R)*((1392340654334763*cos(q1R))/2251799813685248 + (398031123528767*sin(q1R))/562949953421312)))/36893488147419103232 - sin(q3R)*((3480118470877607344838997022995*sin(q2R))/10141204801825835211973625643008 + cos(q2R)*((1392340654334763*cos(q1R))/2251799813685248 + (398031123528767*sin(q1R))/562949953421312) - (7514214926474921*sin(q2R)*((398031123528767*cos(q1R))/562949953421312 - (1392340654334763*sin(q1R))/2251799813685248))/36893488147419103232) + (9007199067919185*cos(q3R)*((3585145564851136108341178694895*cos(q1R))/5070602400912917605986812821504 - (12541089443950065443620820128155*sin(q1R))/20282409603651670423947251286016 + 2903273033334964234439083875867/41538374868278621028243970633760768))/9007199254740992))/36893488147419103232 + ((7514214926474921*cos(q4R))/36893488147419103232 + (4503599440548691*sin(q4R))/4503599627370496)*(cos(q3R)*((3480118470877607344838997022995*sin(q2R))/10141204801825835211973625643008 + cos(q2R)*((1392340654334763*cos(q1R))/2251799813685248 + (398031123528767*sin(q1R))/562949953421312) - (7514214926474921*sin(q2R)*((398031123528767*cos(q1R))/562949953421312 - (1392340654334763*sin(q1R))/2251799813685248))/36893488147419103232) + (7514214926474921*sin(q3R)*((7514214926474921*cos(q2R)*((398031123528767*cos(q1R))/562949953421312 - (1392340654334763*sin(q1R))/2251799813685248))/36893488147419103232 - (3480118470877607344838997022995*cos(q2R))/10141204801825835211973625643008 + sin(q2R)*((1392340654334763*cos(q1R))/2251799813685248 + (398031123528767*sin(q1R))/562949953421312)))/36893488147419103232 + (9007199067919185*sin(q3R)*((3585145564851136108341178694895*cos(q1R))/5070602400912917605986812821504 - (12541089443950065443620820128155*sin(q1R))/20282409603651670423947251286016 + 2903273033334964234439083875867/41538374868278621028243970633760768))/9007199254740992) - ((9007199067919185*cos(q4R))/9007199254740992 - (234819211581865*sin(q4R))/1152921504606846976)*((26939554316989768830159504461322709929728228295*cos(q1R))/187072209578355573530071658587684226515959365500928 + (31346119847137124244279794758002175024246659075*cos(q2R))/91343852333181432387730302044767688728495783936 - (94236441493986648894942587121893377357613500755*sin(q1R))/748288838313422294120286634350736906063837462003712 - (67682029681889335677290557259385*cos(q2R)*((398031123528767*cos(q1R))/562949953421312 - (1392340654334763*sin(q1R))/2251799813685248))/332306998946228968225951765070086144 - (9007199067919185*sin(q2R)*((1392340654334763*cos(q1R))/2251799813685248 + (398031123528767*sin(q1R))/562949953421312))/9007199254740992 + 21815817562717709140362801846989786744252631507/1532495540865888858358347027150309183618739122183602176)) - (7514214926474921*sin(q5R)*(((4503599440548691*cos(q4R))/4503599627370496 - (7514214926474921*sin(q4R))/36893488147419103232)*(cos(q3R)*((3480118470877607344838997022995*sin(q2R))/10141204801825835211973625643008 + cos(q2R)*((1392340654334763*cos(q1R))/2251799813685248 + (398031123528767*sin(q1R))/562949953421312) - (7514214926474921*sin(q2R)*((398031123528767*cos(q1R))/562949953421312 - (1392340654334763*sin(q1R))/2251799813685248))/36893488147419103232) + (7514214926474921*sin(q3R)*((7514214926474921*cos(q2R)*((398031123528767*cos(q1R))/562949953421312 - (1392340654334763*sin(q1R))/2251799813685248))/36893488147419103232 - (3480118470877607344838997022995*cos(q2R))/10141204801825835211973625643008 + sin(q2R)*((1392340654334763*cos(q1R))/2251799813685248 + (398031123528767*sin(q1R))/562949953421312)))/36893488147419103232 + (9007199067919185*sin(q3R)*((3585145564851136108341178694895*cos(q1R))/5070602400912917605986812821504 - (12541089443950065443620820128155*sin(q1R))/20282409603651670423947251286016 + 2903273033334964234439083875867/41538374868278621028243970633760768))/9007199254740992) + ((234819211581865*cos(q4R))/1152921504606846976 + (9007199067919185*sin(q4R))/9007199254740992)*((26939554316989768830159504461322709929728228295*cos(q1R))/187072209578355573530071658587684226515959365500928 + (31346119847137124244279794758002175024246659075*cos(q2R))/91343852333181432387730302044767688728495783936 - (94236441493986648894942587121893377357613500755*sin(q1R))/748288838313422294120286634350736906063837462003712 - (67682029681889335677290557259385*cos(q2R)*((398031123528767*cos(q1R))/562949953421312 - (1392340654334763*sin(q1R))/2251799813685248))/332306998946228968225951765070086144 - (9007199067919185*sin(q2R)*((1392340654334763*cos(q1R))/2251799813685248 + (398031123528767*sin(q1R))/562949953421312))/9007199254740992 + 21815817562717709140362801846989786744252631507/1532495540865888858358347027150309183618739122183602176) + (7514214926474921*cos(q4R)*((7514214926474921*cos(q3R)*((7514214926474921*cos(q2R)*((398031123528767*cos(q1R))/562949953421312 - (1392340654334763*sin(q1R))/2251799813685248))/36893488147419103232 - (3480118470877607344838997022995*cos(q2R))/10141204801825835211973625643008 + sin(q2R)*((1392340654334763*cos(q1R))/2251799813685248 + (398031123528767*sin(q1R))/562949953421312)))/36893488147419103232 - sin(q3R)*((3480118470877607344838997022995*sin(q2R))/10141204801825835211973625643008 + cos(q2R)*((1392340654334763*cos(q1R))/2251799813685248 + (398031123528767*sin(q1R))/562949953421312) - (7514214926474921*sin(q2R)*((398031123528767*cos(q1R))/562949953421312 - (1392340654334763*sin(q1R))/2251799813685248))/36893488147419103232) + (9007199067919185*cos(q3R)*((3585145564851136108341178694895*cos(q1R))/5070602400912917605986812821504 - (12541089443950065443620820128155*sin(q1R))/20282409603651670423947251286016 + 2903273033334964234439083875867/41538374868278621028243970633760768))/9007199254740992))/36893488147419103232))/36893488147419103232 + (9007199067919185*sin(q5R)*((42218993040650622024393554167529407181397382817729417611526625*cos(q1R))/7067388259113537318333190002971674063309935587502475832486424805170479104 + (49124851885283889459147163519037433596494512994900179139213125*cos(q2R))/3450873173395281893717377931138512726225554486085193277581262111899648 - (147684984717849177105467939785270041851792306559769220895307125*sin(q1R))/28269553036454149273332760011886696253239742350009903329945699220681916416 - (67682029681889335677290557259385*cos(q3R)*((7514214926474921*cos(q2R)*((398031123528767*cos(q1R))/562949953421312 - (1392340654334763*sin(q1R))/2251799813685248))/36893488147419103232 - (3480118470877607344838997022995*cos(q2R))/10141204801825835211973625643008 + sin(q2R)*((1392340654334763*cos(q1R))/2251799813685248 + (398031123528767*sin(q1R))/562949953421312)))/332306998946228968225951765070086144 + (234819211581865*cos(q3R)*((3480118470877607344838997022995*sin(q2R))/10141204801825835211973625643008 + cos(q2R)*((1392340654334763*cos(q1R))/2251799813685248 + (398031123528767*sin(q1R))/562949953421312) - (7514214926474921*sin(q2R)*((398031123528767*cos(q1R))/562949953421312 - (1392340654334763*sin(q1R))/2251799813685248))/36893488147419103232))/1152921504606846976 + (1764482024691522628700660907665*sin(q3R)*((7514214926474921*cos(q2R)*((398031123528767*cos(q1R))/562949953421312 - (1392340654334763*sin(q1R))/2251799813685248))/36893488147419103232 - (3480118470877607344838997022995*cos(q2R))/10141204801825835211973625643008 + sin(q2R)*((1392340654334763*cos(q1R))/2251799813685248 + (398031123528767*sin(q1R))/562949953421312)))/42535295865117307932921825928971026432 + (9007199067919185*sin(q3R)*((3480118470877607344838997022995*sin(q2R))/10141204801825835211973625643008 + cos(q2R)*((1392340654334763*cos(q1R))/2251799813685248 + (398031123528767*sin(q1R))/562949953421312) - (7514214926474921*sin(q2R)*((398031123528767*cos(q1R))/562949953421312 - (1392340654334763*sin(q1R))/2251799813685248))/36893488147419103232))/9007199254740992 - (106069577339469832923929692356850887620017617375*cos(q2R)*((398031123528767*cos(q1R))/562949953421312 - (1392340654334763*sin(q1R))/2251799813685248))/12554203470773361527671578846415332832204710888928069025792 - (81129635049124235038645691064225*cos(q3R)*((3585145564851136108341178694895*cos(q1R))/5070602400912917605986812821504 - (12541089443950065443620820128155*sin(q1R))/20282409603651670423947251286016 + 2903273033334964234439083875867/41538374868278621028243970633760768))/81129638414606681695789005144064 - (14115856197532180673579726082375*sin(q2R)*((1392340654334763*cos(q1R))/2251799813685248 + (398031123528767*sin(q1R))/562949953421312))/340282366920938463463374607431768211456 + (2115063383689692319117831580025*sin(q3R)*((3585145564851136108341178694895*cos(q1R))/5070602400912917605986812821504 - (12541089443950065443620820128155*sin(q1R))/20282409603651670423947251286016 + 2903273033334964234439083875867/41538374868278621028243970633760768))/10384593717069655257060992658440192 + 34189201462609793352471527538206775118278208232606556159508725/57896044618658097711785492504343953926634992332820282019728792003956564819968))/9007199254740992))/1000 + (48638874966763599*cos(q6R)*((317242587686797715160741214886285987125185037094314753690999507962888586271625*cos(q1R))/260740604970814219042361048116400404614587954389239840081425977517360806369707098391474864128 + (369134695297269865703468593411141398729137707824460658574000083747077986538125*cos(q2R))/127314748520905380391777855525586135065716774604121015664758778084648831235208544136462336 - (1109736716583082885849910318389051322854142663349680644790580040185967905112125*sin(q1R))/1042962419883256876169444192465601618458351817556959360325703910069443225478828393565899456512 - (508577317689771495245073589786522929324694383585*cos(q3R)*((7514214926474921*cos(q2R)*((398031123528767*cos(q1R))/562949953421312 - (1392340654334763*sin(q1R))/2251799813685248))/36893488147419103232 - (3480118470877607344838997022995*cos(q2R))/10141204801825835211973625643008 + sin(q2R)*((1392340654334763*cos(q1R))/2251799813685248 + (398031123528767*sin(q1R))/562949953421312)))/12259964326927110866866776217202473468949912977468817408 + (1764482024691522628700660907665*cos(q3R)*((3480118470877607344838997022995*sin(q2R))/10141204801825835211973625643008 + cos(q2R)*((1392340654334763*cos(q1R))/2251799813685248 + (398031123528767*sin(q1R))/562949953421312) - (7514214926474921*sin(q2R)*((398031123528767*cos(q1R))/562949953421312 - (1392340654334763*sin(q1R))/2251799813685248))/36893488147419103232))/42535295865117307932921825928971026432 + (13258697167433729449897784796786197386719169465*sin(q3R)*((7514214926474921*cos(q2R)*((398031123528767*cos(q1R))/562949953421312 - (1392340654334763*sin(q1R))/2251799813685248))/36893488147419103232 - (3480118470877607344838997022995*cos(q2R))/10141204801825835211973625643008 + sin(q2R)*((1392340654334763*cos(q1R))/2251799813685248 + (398031123528767*sin(q1R))/562949953421312)))/1569275433846670190958947355801916604025588861116008628224 + (67682029681889335677290557259385*sin(q3R)*((3480118470877607344838997022995*sin(q2R))/10141204801825835211973625643008 + cos(q2R)*((1392340654334763*cos(q1R))/2251799813685248 + (398031123528767*sin(q1R))/562949953421312) - (7514214926474921*sin(q2R)*((398031123528767*cos(q1R))/562949953421312 - (1392340654334763*sin(q1R))/2251799813685248))/36893488147419103232))/332306998946228968225951765070086144 - (797029601289130257223357069404502671534492977261568326111352375*cos(q2R)*((398031123528767*cos(q1R))/562949953421312 - (1392340654334763*sin(q1R))/2251799813685248))/463168356949264781694283940034751631413079938662562256157830336031652518559744 - (609625514665592237562888769449172969868262801225*cos(q3R)*((3585145564851136108341178694895*cos(q1R))/5070602400912917605986812821504 - (12541089443950065443620820128155*sin(q1R))/20282409603651670423947251286016 + 2903273033334964234439083875867/41538374868278621028243970633760768))/2993155353253689176481146537402947624255349848014848 + (9007199067919185*((4503599440548691*cos(q4R))/4503599627370496 - (7514214926474921*sin(q4R))/36893488147419103232)*(cos(q3R)*((3480118470877607344838997022995*sin(q2R))/10141204801825835211973625643008 + cos(q2R)*((1392340654334763*cos(q1R))/2251799813685248 + (398031123528767*sin(q1R))/562949953421312) - (7514214926474921*sin(q2R)*((398031123528767*cos(q1R))/562949953421312 - (1392340654334763*sin(q1R))/2251799813685248))/36893488147419103232) + (7514214926474921*sin(q3R)*((7514214926474921*cos(q2R)*((398031123528767*cos(q1R))/562949953421312 - (1392340654334763*sin(q1R))/2251799813685248))/36893488147419103232 - (3480118470877607344838997022995*cos(q2R))/10141204801825835211973625643008 + sin(q2R)*((1392340654334763*cos(q1R))/2251799813685248 + (398031123528767*sin(q1R))/562949953421312)))/36893488147419103232 + (9007199067919185*sin(q3R)*((3585145564851136108341178694895*cos(q1R))/5070602400912917605986812821504 - (12541089443950065443620820128155*sin(q1R))/20282409603651670423947251286016 + 2903273033334964234439083875867/41538374868278621028243970633760768))/9007199254740992))/9007199254740992 - (106069577339469832923929692356850887620017617375*sin(q2R)*((1392340654334763*cos(q1R))/2251799813685248 + (398031123528767*sin(q1R))/562949953421312))/12554203470773361527671578846415332832204710888928069025792 + (15893040848161638993908057577265778144967053025*sin(q3R)*((3585145564851136108341178694895*cos(q1R))/5070602400912917605986812821504 - (12541089443950065443620820128155*sin(q1R))/20282409603651670423947251286016 + 2903273033334964234439083875867/41538374868278621028243970633760768))/383123885216472214589586756787577295904684780545900544 + (9007199067919185*((234819211581865*cos(q4R))/1152921504606846976 + (9007199067919185*sin(q4R))/9007199254740992)*((26939554316989768830159504461322709929728228295*cos(q1R))/187072209578355573530071658587684226515959365500928 + (31346119847137124244279794758002175024246659075*cos(q2R))/91343852333181432387730302044767688728495783936 - (94236441493986648894942587121893377357613500755*sin(q1R))/748288838313422294120286634350736906063837462003712 - (67682029681889335677290557259385*cos(q2R)*((398031123528767*cos(q1R))/562949953421312 - (1392340654334763*sin(q1R))/2251799813685248))/332306998946228968225951765070086144 - (9007199067919185*sin(q2R)*((1392340654334763*cos(q1R))/2251799813685248 + (398031123528767*sin(q1R))/562949953421312))/9007199254740992 + 21815817562717709140362801846989786744252631507/1532495540865888858358347027150309183618739122183602176))/9007199254740992 + (67682029681889335677290557259385*cos(q4R)*((7514214926474921*cos(q3R)*((7514214926474921*cos(q2R)*((398031123528767*cos(q1R))/562949953421312 - (1392340654334763*sin(q1R))/2251799813685248))/36893488147419103232 - (3480118470877607344838997022995*cos(q2R))/10141204801825835211973625643008 + sin(q2R)*((1392340654334763*cos(q1R))/2251799813685248 + (398031123528767*sin(q1R))/562949953421312)))/36893488147419103232 - sin(q3R)*((3480118470877607344838997022995*sin(q2R))/10141204801825835211973625643008 + cos(q2R)*((1392340654334763*cos(q1R))/2251799813685248 + (398031123528767*sin(q1R))/562949953421312) - (7514214926474921*sin(q2R)*((398031123528767*cos(q1R))/562949953421312 - (1392340654334763*sin(q1R))/2251799813685248))/36893488147419103232) + (9007199067919185*cos(q3R)*((3585145564851136108341178694895*cos(q1R))/5070602400912917605986812821504 - (12541089443950065443620820128155*sin(q1R))/20282409603651670423947251286016 + 2903273033334964234439083875867/41538374868278621028243970633760768))/9007199254740992))/332306998946228968225951765070086144 + 256905007954600709870741236886362515198064227567936069111275436480059393185725/2135987035920910082395021706169552114602704522356652769947041607822219725780640550022962086936576))/1801439850948198400, 0; (81222263116692158804177042061221826384594597321566869716687*((4503599440548691*cos(q4R))/4503599627370496 - (7514214926474921*sin(q4R))/36893488147419103232)*((9007199067919185*sin(q3R)*((10914283902180054573281797610715*cos(q1R))/20282409603651670423947251286016 - (28359221366286827792295350160645*sin(q1R))/40564819207303340847894502572032))/9007199254740992 + cos(q3R)*(cos(q2R)*((3148506117433717*cos(q1R))/4503599627370496 + (1211728953682539*sin(q1R))/2251799813685248) - (7514214926474921*sin(q2R)*((1211728953682539*cos(q1R))/2251799813685248 - (3148506117433717*sin(q1R))/4503599627370496))/36893488147419103232) + (7514214926474921*sin(q3R)*((7514214926474921*cos(q2R)*((1211728953682539*cos(q1R))/2251799813685248 - (3148506117433717*sin(q1R))/4503599627370496))/36893488147419103232 + sin(q2R)*((3148506117433717*cos(q1R))/4503599627370496 + (1211728953682539*sin(q1R))/2251799813685248)))/36893488147419103232))/306499108173177771671669405430061836723747824436720435200000 - (229014705556396818278503769072946954655822455216536876552533377799556736621320936323753181652197846160461653487964587881416342571260633*sin(q1R))/14196068833898572081041480622812588561594557825924180864872855452746861095964803189964668959253194639858643000122386287764347688058880000 - (148930196498699323999461223284752477897935758922663835370060473617773193914687139045748299910261535468144466000731355074781576713920889*cos(q1R))/7098034416949286040520740311406294280797278912962090432436427726373430547982401594982334479626597319929321500061193143882173844029440000 + (81*((7514214926474921*cos(q4R))/36893488147419103232 + (4503599440548691*sin(q4R))/4503599627370496)*((9007199067919185*sin(q3R)*((10914283902180054573281797610715*cos(q1R))/20282409603651670423947251286016 - (28359221366286827792295350160645*sin(q1R))/40564819207303340847894502572032))/9007199254740992 + cos(q3R)*(cos(q2R)*((3148506117433717*cos(q1R))/4503599627370496 + (1211728953682539*sin(q1R))/2251799813685248) - (7514214926474921*sin(q2R)*((1211728953682539*cos(q1R))/2251799813685248 - (3148506117433717*sin(q1R))/4503599627370496))/36893488147419103232) + (7514214926474921*sin(q3R)*((7514214926474921*cos(q2R)*((1211728953682539*cos(q1R))/2251799813685248 - (3148506117433717*sin(q1R))/4503599627370496))/36893488147419103232 + sin(q2R)*((3148506117433717*cos(q1R))/4503599627370496 + (1211728953682539*sin(q1R))/2251799813685248)))/36893488147419103232))/2000 + (2436553109258773196144549622003023*cos(q6R)*((7514214926474921*cos(q5R)*(((4503599440548691*cos(q4R))/4503599627370496 - (7514214926474921*sin(q4R))/36893488147419103232)*((9007199067919185*sin(q3R)*((10914283902180054573281797610715*cos(q1R))/20282409603651670423947251286016 - (28359221366286827792295350160645*sin(q1R))/40564819207303340847894502572032))/9007199254740992 + cos(q3R)*(cos(q2R)*((3148506117433717*cos(q1R))/4503599627370496 + (1211728953682539*sin(q1R))/2251799813685248) - (7514214926474921*sin(q2R)*((1211728953682539*cos(q1R))/2251799813685248 - (3148506117433717*sin(q1R))/4503599627370496))/36893488147419103232) + (7514214926474921*sin(q3R)*((7514214926474921*cos(q2R)*((1211728953682539*cos(q1R))/2251799813685248 - (3148506117433717*sin(q1R))/4503599627370496))/36893488147419103232 + sin(q2R)*((3148506117433717*cos(q1R))/4503599627370496 + (1211728953682539*sin(q1R))/2251799813685248)))/36893488147419103232) - ((234819211581865*cos(q4R))/1152921504606846976 + (9007199067919185*sin(q4R))/9007199254740992)*((213097284493758984364555654519459856780913684045*sin(q1R))/1496577676626844588240573268701473812127674924007424 - (82012275009546312639155898108543355135168378515*cos(q1R))/748288838313422294120286634350736906063837462003712 + (67682029681889335677290557259385*cos(q2R)*((1211728953682539*cos(q1R))/2251799813685248 - (3148506117433717*sin(q1R))/4503599627370496))/332306998946228968225951765070086144 + (9007199067919185*sin(q2R)*((3148506117433717*cos(q1R))/4503599627370496 + (1211728953682539*sin(q1R))/2251799813685248))/9007199254740992) + (7514214926474921*cos(q4R)*((9007199067919185*cos(q3R)*((10914283902180054573281797610715*cos(q1R))/20282409603651670423947251286016 - (28359221366286827792295350160645*sin(q1R))/40564819207303340847894502572032))/9007199254740992 + (7514214926474921*cos(q3R)*((7514214926474921*cos(q2R)*((1211728953682539*cos(q1R))/2251799813685248 - (3148506117433717*sin(q1R))/4503599627370496))/36893488147419103232 + sin(q2R)*((3148506117433717*cos(q1R))/4503599627370496 + (1211728953682539*sin(q1R))/2251799813685248)))/36893488147419103232 - sin(q3R)*(cos(q2R)*((3148506117433717*cos(q1R))/4503599627370496 + (1211728953682539*sin(q1R))/2251799813685248) - (7514214926474921*sin(q2R)*((1211728953682539*cos(q1R))/2251799813685248 - (3148506117433717*sin(q1R))/4503599627370496))/36893488147419103232)))/36893488147419103232))/36893488147419103232 - (9007199067919185*cos(q5R)*((128527577967104929471702655059245076724477257328642562920515125*cos(q1R))/28269553036454149273332760011886696253239742350009903329945699220681916416 - (333960713126929533372903469589741180908441336378844163830032875*sin(q1R))/56539106072908298546665520023773392506479484700019806659891398441363832832 - (106069577339469832923929692356850887620017617375*cos(q2R)*((1211728953682539*cos(q1R))/2251799813685248 - (3148506117433717*sin(q1R))/4503599627370496))/12554203470773361527671578846415332832204710888928069025792 - (14115856197532180673579726082375*sin(q2R)*((3148506117433717*cos(q1R))/4503599627370496 + (1211728953682539*sin(q1R))/2251799813685248))/340282366920938463463374607431768211456 - (81129635049124235038645691064225*cos(q3R)*((10914283902180054573281797610715*cos(q1R))/20282409603651670423947251286016 - (28359221366286827792295350160645*sin(q1R))/40564819207303340847894502572032))/81129638414606681695789005144064 + (2115063383689692319117831580025*sin(q3R)*((10914283902180054573281797610715*cos(q1R))/20282409603651670423947251286016 - (28359221366286827792295350160645*sin(q1R))/40564819207303340847894502572032))/10384593717069655257060992658440192 + (234819211581865*cos(q3R)*(cos(q2R)*((3148506117433717*cos(q1R))/4503599627370496 + (1211728953682539*sin(q1R))/2251799813685248) - (7514214926474921*sin(q2R)*((1211728953682539*cos(q1R))/2251799813685248 - (3148506117433717*sin(q1R))/4503599627370496))/36893488147419103232))/1152921504606846976 - (67682029681889335677290557259385*cos(q3R)*((7514214926474921*cos(q2R)*((1211728953682539*cos(q1R))/2251799813685248 - (3148506117433717*sin(q1R))/4503599627370496))/36893488147419103232 + sin(q2R)*((3148506117433717*cos(q1R))/4503599627370496 + (1211728953682539*sin(q1R))/2251799813685248)))/332306998946228968225951765070086144 + (9007199067919185*sin(q3R)*(cos(q2R)*((3148506117433717*cos(q1R))/4503599627370496 + (1211728953682539*sin(q1R))/2251799813685248) - (7514214926474921*sin(q2R)*((1211728953682539*cos(q1R))/2251799813685248 - (3148506117433717*sin(q1R))/4503599627370496))/36893488147419103232))/9007199254740992 + (1764482024691522628700660907665*sin(q3R)*((7514214926474921*cos(q2R)*((1211728953682539*cos(q1R))/2251799813685248 - (3148506117433717*sin(q1R))/4503599627370496))/36893488147419103232 + sin(q2R)*((3148506117433717*cos(q1R))/4503599627370496 + (1211728953682539*sin(q1R))/2251799813685248)))/42535295865117307932921825928971026432))/9007199254740992 + sin(q5R)*(((7514214926474921*cos(q4R))/36893488147419103232 + (4503599440548691*sin(q4R))/4503599627370496)*((9007199067919185*sin(q3R)*((10914283902180054573281797610715*cos(q1R))/20282409603651670423947251286016 - (28359221366286827792295350160645*sin(q1R))/40564819207303340847894502572032))/9007199254740992 + cos(q3R)*(cos(q2R)*((3148506117433717*cos(q1R))/4503599627370496 + (1211728953682539*sin(q1R))/2251799813685248) - (7514214926474921*sin(q2R)*((1211728953682539*cos(q1R))/2251799813685248 - (3148506117433717*sin(q1R))/4503599627370496))/36893488147419103232) + (7514214926474921*sin(q3R)*((7514214926474921*cos(q2R)*((1211728953682539*cos(q1R))/2251799813685248 - (3148506117433717*sin(q1R))/4503599627370496))/36893488147419103232 + sin(q2R)*((3148506117433717*cos(q1R))/4503599627370496 + (1211728953682539*sin(q1R))/2251799813685248)))/36893488147419103232) + ((9007199067919185*cos(q4R))/9007199254740992 - (234819211581865*sin(q4R))/1152921504606846976)*((213097284493758984364555654519459856780913684045*sin(q1R))/1496577676626844588240573268701473812127674924007424 - (82012275009546312639155898108543355135168378515*cos(q1R))/748288838313422294120286634350736906063837462003712 + (67682029681889335677290557259385*cos(q2R)*((1211728953682539*cos(q1R))/2251799813685248 - (3148506117433717*sin(q1R))/4503599627370496))/332306998946228968225951765070086144 + (9007199067919185*sin(q2R)*((3148506117433717*cos(q1R))/4503599627370496 + (1211728953682539*sin(q1R))/2251799813685248))/9007199254740992) + (7514214926474921*sin(q4R)*((9007199067919185*cos(q3R)*((10914283902180054573281797610715*cos(q1R))/20282409603651670423947251286016 - (28359221366286827792295350160645*sin(q1R))/40564819207303340847894502572032))/9007199254740992 + (7514214926474921*cos(q3R)*((7514214926474921*cos(q2R)*((1211728953682539*cos(q1R))/2251799813685248 - (3148506117433717*sin(q1R))/4503599627370496))/36893488147419103232 + sin(q2R)*((3148506117433717*cos(q1R))/4503599627370496 + (1211728953682539*sin(q1R))/2251799813685248)))/36893488147419103232 - sin(q3R)*(cos(q2R)*((3148506117433717*cos(q1R))/4503599627370496 + (1211728953682539*sin(q1R))/2251799813685248) - (7514214926474921*sin(q2R)*((1211728953682539*cos(q1R))/2251799813685248 - (3148506117433717*sin(q1R))/4503599627370496))/36893488147419103232)))/36893488147419103232)))/332306998946228968225951765070086144000 + (81*((9007199067919185*cos(q4R))/9007199254740992 - (234819211581865*sin(q4R))/1152921504606846976)*((213097284493758984364555654519459856780913684045*sin(q1R))/1496577676626844588240573268701473812127674924007424 - (82012275009546312639155898108543355135168378515*cos(q1R))/748288838313422294120286634350736906063837462003712 + (67682029681889335677290557259385*cos(q2R)*((1211728953682539*cos(q1R))/2251799813685248 - (3148506117433717*sin(q1R))/4503599627370496))/332306998946228968225951765070086144 + (9007199067919185*sin(q2R)*((3148506117433717*cos(q1R))/4503599627370496 + (1211728953682539*sin(q1R))/2251799813685248))/9007199254740992))/2000 - (81222263116692158804177042061221826384594597321566869716687*((234819211581865*cos(q4R))/1152921504606846976 + (9007199067919185*sin(q4R))/9007199254740992)*((213097284493758984364555654519459856780913684045*sin(q1R))/1496577676626844588240573268701473812127674924007424 - (82012275009546312639155898108543355135168378515*cos(q1R))/748288838313422294120286634350736906063837462003712 + (67682029681889335677290557259385*cos(q2R)*((1211728953682539*cos(q1R))/2251799813685248 - (3148506117433717*sin(q1R))/4503599627370496))/332306998946228968225951765070086144 + (9007199067919185*sin(q2R)*((3148506117433717*cos(q1R))/4503599627370496 + (1211728953682539*sin(q1R))/2251799813685248))/9007199254740992))/306499108173177771671669405430061836723747824436720435200000 + (27*cos(q6R)*(cos(q5R)*(((7514214926474921*cos(q4R))/36893488147419103232 + (4503599440548691*sin(q4R))/4503599627370496)*((9007199067919185*sin(q3R)*((10914283902180054573281797610715*cos(q1R))/20282409603651670423947251286016 - (28359221366286827792295350160645*sin(q1R))/40564819207303340847894502572032))/9007199254740992 + cos(q3R)*(cos(q2R)*((3148506117433717*cos(q1R))/4503599627370496 + (1211728953682539*sin(q1R))/2251799813685248) - (7514214926474921*sin(q2R)*((1211728953682539*cos(q1R))/2251799813685248 - (3148506117433717*sin(q1R))/4503599627370496))/36893488147419103232) + (7514214926474921*sin(q3R)*((7514214926474921*cos(q2R)*((1211728953682539*cos(q1R))/2251799813685248 - (3148506117433717*sin(q1R))/4503599627370496))/36893488147419103232 + sin(q2R)*((3148506117433717*cos(q1R))/4503599627370496 + (1211728953682539*sin(q1R))/2251799813685248)))/36893488147419103232) + ((9007199067919185*cos(q4R))/9007199254740992 - (234819211581865*sin(q4R))/1152921504606846976)*((213097284493758984364555654519459856780913684045*sin(q1R))/1496577676626844588240573268701473812127674924007424 - (82012275009546312639155898108543355135168378515*cos(q1R))/748288838313422294120286634350736906063837462003712 + (67682029681889335677290557259385*cos(q2R)*((1211728953682539*cos(q1R))/2251799813685248 - (3148506117433717*sin(q1R))/4503599627370496))/332306998946228968225951765070086144 + (9007199067919185*sin(q2R)*((3148506117433717*cos(q1R))/4503599627370496 + (1211728953682539*sin(q1R))/2251799813685248))/9007199254740992) + (7514214926474921*sin(q4R)*((9007199067919185*cos(q3R)*((10914283902180054573281797610715*cos(q1R))/20282409603651670423947251286016 - (28359221366286827792295350160645*sin(q1R))/40564819207303340847894502572032))/9007199254740992 + (7514214926474921*cos(q3R)*((7514214926474921*cos(q2R)*((1211728953682539*cos(q1R))/2251799813685248 - (3148506117433717*sin(q1R))/4503599627370496))/36893488147419103232 + sin(q2R)*((3148506117433717*cos(q1R))/4503599627370496 + (1211728953682539*sin(q1R))/2251799813685248)))/36893488147419103232 - sin(q3R)*(cos(q2R)*((3148506117433717*cos(q1R))/4503599627370496 + (1211728953682539*sin(q1R))/2251799813685248) - (7514214926474921*sin(q2R)*((1211728953682539*cos(q1R))/2251799813685248 - (3148506117433717*sin(q1R))/4503599627370496))/36893488147419103232)))/36893488147419103232) - (7514214926474921*sin(q5R)*(((4503599440548691*cos(q4R))/4503599627370496 - (7514214926474921*sin(q4R))/36893488147419103232)*((9007199067919185*sin(q3R)*((10914283902180054573281797610715*cos(q1R))/20282409603651670423947251286016 - (28359221366286827792295350160645*sin(q1R))/40564819207303340847894502572032))/9007199254740992 + cos(q3R)*(cos(q2R)*((3148506117433717*cos(q1R))/4503599627370496 + (1211728953682539*sin(q1R))/2251799813685248) - (7514214926474921*sin(q2R)*((1211728953682539*cos(q1R))/2251799813685248 - (3148506117433717*sin(q1R))/4503599627370496))/36893488147419103232) + (7514214926474921*sin(q3R)*((7514214926474921*cos(q2R)*((1211728953682539*cos(q1R))/2251799813685248 - (3148506117433717*sin(q1R))/4503599627370496))/36893488147419103232 + sin(q2R)*((3148506117433717*cos(q1R))/4503599627370496 + (1211728953682539*sin(q1R))/2251799813685248)))/36893488147419103232) - ((234819211581865*cos(q4R))/1152921504606846976 + (9007199067919185*sin(q4R))/9007199254740992)*((213097284493758984364555654519459856780913684045*sin(q1R))/1496577676626844588240573268701473812127674924007424 - (82012275009546312639155898108543355135168378515*cos(q1R))/748288838313422294120286634350736906063837462003712 + (67682029681889335677290557259385*cos(q2R)*((1211728953682539*cos(q1R))/2251799813685248 - (3148506117433717*sin(q1R))/4503599627370496))/332306998946228968225951765070086144 + (9007199067919185*sin(q2R)*((3148506117433717*cos(q1R))/4503599627370496 + (1211728953682539*sin(q1R))/2251799813685248))/9007199254740992) + (7514214926474921*cos(q4R)*((9007199067919185*cos(q3R)*((10914283902180054573281797610715*cos(q1R))/20282409603651670423947251286016 - (28359221366286827792295350160645*sin(q1R))/40564819207303340847894502572032))/9007199254740992 + (7514214926474921*cos(q3R)*((7514214926474921*cos(q2R)*((1211728953682539*cos(q1R))/2251799813685248 - (3148506117433717*sin(q1R))/4503599627370496))/36893488147419103232 + sin(q2R)*((3148506117433717*cos(q1R))/4503599627370496 + (1211728953682539*sin(q1R))/2251799813685248)))/36893488147419103232 - sin(q3R)*(cos(q2R)*((3148506117433717*cos(q1R))/4503599627370496 + (1211728953682539*sin(q1R))/2251799813685248) - (7514214926474921*sin(q2R)*((1211728953682539*cos(q1R))/2251799813685248 - (3148506117433717*sin(q1R))/4503599627370496))/36893488147419103232)))/36893488147419103232))/36893488147419103232 + (9007199067919185*sin(q5R)*((128527577967104929471702655059245076724477257328642562920515125*cos(q1R))/28269553036454149273332760011886696253239742350009903329945699220681916416 - (333960713126929533372903469589741180908441336378844163830032875*sin(q1R))/56539106072908298546665520023773392506479484700019806659891398441363832832 - (106069577339469832923929692356850887620017617375*cos(q2R)*((1211728953682539*cos(q1R))/2251799813685248 - (3148506117433717*sin(q1R))/4503599627370496))/12554203470773361527671578846415332832204710888928069025792 - (14115856197532180673579726082375*sin(q2R)*((3148506117433717*cos(q1R))/4503599627370496 + (1211728953682539*sin(q1R))/2251799813685248))/340282366920938463463374607431768211456 - (81129635049124235038645691064225*cos(q3R)*((10914283902180054573281797610715*cos(q1R))/20282409603651670423947251286016 - (28359221366286827792295350160645*sin(q1R))/40564819207303340847894502572032))/81129638414606681695789005144064 + (2115063383689692319117831580025*sin(q3R)*((10914283902180054573281797610715*cos(q1R))/20282409603651670423947251286016 - (28359221366286827792295350160645*sin(q1R))/40564819207303340847894502572032))/10384593717069655257060992658440192 + (234819211581865*cos(q3R)*(cos(q2R)*((3148506117433717*cos(q1R))/4503599627370496 + (1211728953682539*sin(q1R))/2251799813685248) - (7514214926474921*sin(q2R)*((1211728953682539*cos(q1R))/2251799813685248 - (3148506117433717*sin(q1R))/4503599627370496))/36893488147419103232))/1152921504606846976 - (67682029681889335677290557259385*cos(q3R)*((7514214926474921*cos(q2R)*((1211728953682539*cos(q1R))/2251799813685248 - (3148506117433717*sin(q1R))/4503599627370496))/36893488147419103232 + sin(q2R)*((3148506117433717*cos(q1R))/4503599627370496 + (1211728953682539*sin(q1R))/2251799813685248)))/332306998946228968225951765070086144 + (9007199067919185*sin(q3R)*(cos(q2R)*((3148506117433717*cos(q1R))/4503599627370496 + (1211728953682539*sin(q1R))/2251799813685248) - (7514214926474921*sin(q2R)*((1211728953682539*cos(q1R))/2251799813685248 - (3148506117433717*sin(q1R))/4503599627370496))/36893488147419103232))/9007199254740992 + (1764482024691522628700660907665*sin(q3R)*((7514214926474921*cos(q2R)*((1211728953682539*cos(q1R))/2251799813685248 - (3148506117433717*sin(q1R))/4503599627370496))/36893488147419103232 + sin(q2R)*((3148506117433717*cos(q1R))/4503599627370496 + (1211728953682539*sin(q1R))/2251799813685248)))/42535295865117307932921825928971026432))/9007199254740992))/1000 + (202883803014822867*sin(q6R)*((7514214926474921*cos(q5R)*(((4503599440548691*cos(q4R))/4503599627370496 - (7514214926474921*sin(q4R))/36893488147419103232)*((9007199067919185*sin(q3R)*((10914283902180054573281797610715*cos(q1R))/20282409603651670423947251286016 - (28359221366286827792295350160645*sin(q1R))/40564819207303340847894502572032))/9007199254740992 + cos(q3R)*(cos(q2R)*((3148506117433717*cos(q1R))/4503599627370496 + (1211728953682539*sin(q1R))/2251799813685248) - (7514214926474921*sin(q2R)*((1211728953682539*cos(q1R))/2251799813685248 - (3148506117433717*sin(q1R))/4503599627370496))/36893488147419103232) + (7514214926474921*sin(q3R)*((7514214926474921*cos(q2R)*((1211728953682539*cos(q1R))/2251799813685248 - (3148506117433717*sin(q1R))/4503599627370496))/36893488147419103232 + sin(q2R)*((3148506117433717*cos(q1R))/4503599627370496 + (1211728953682539*sin(q1R))/2251799813685248)))/36893488147419103232) - ((234819211581865*cos(q4R))/1152921504606846976 + (9007199067919185*sin(q4R))/9007199254740992)*((213097284493758984364555654519459856780913684045*sin(q1R))/1496577676626844588240573268701473812127674924007424 - (82012275009546312639155898108543355135168378515*cos(q1R))/748288838313422294120286634350736906063837462003712 + (67682029681889335677290557259385*cos(q2R)*((1211728953682539*cos(q1R))/2251799813685248 - (3148506117433717*sin(q1R))/4503599627370496))/332306998946228968225951765070086144 + (9007199067919185*sin(q2R)*((3148506117433717*cos(q1R))/4503599627370496 + (1211728953682539*sin(q1R))/2251799813685248))/9007199254740992) + (7514214926474921*cos(q4R)*((9007199067919185*cos(q3R)*((10914283902180054573281797610715*cos(q1R))/20282409603651670423947251286016 - (28359221366286827792295350160645*sin(q1R))/40564819207303340847894502572032))/9007199254740992 + (7514214926474921*cos(q3R)*((7514214926474921*cos(q2R)*((1211728953682539*cos(q1R))/2251799813685248 - (3148506117433717*sin(q1R))/4503599627370496))/36893488147419103232 + sin(q2R)*((3148506117433717*cos(q1R))/4503599627370496 + (1211728953682539*sin(q1R))/2251799813685248)))/36893488147419103232 - sin(q3R)*(cos(q2R)*((3148506117433717*cos(q1R))/4503599627370496 + (1211728953682539*sin(q1R))/2251799813685248) - (7514214926474921*sin(q2R)*((1211728953682539*cos(q1R))/2251799813685248 - (3148506117433717*sin(q1R))/4503599627370496))/36893488147419103232)))/36893488147419103232))/36893488147419103232 - (9007199067919185*cos(q5R)*((128527577967104929471702655059245076724477257328642562920515125*cos(q1R))/28269553036454149273332760011886696253239742350009903329945699220681916416 - (333960713126929533372903469589741180908441336378844163830032875*sin(q1R))/56539106072908298546665520023773392506479484700019806659891398441363832832 - (106069577339469832923929692356850887620017617375*cos(q2R)*((1211728953682539*cos(q1R))/2251799813685248 - (3148506117433717*sin(q1R))/4503599627370496))/12554203470773361527671578846415332832204710888928069025792 - (14115856197532180673579726082375*sin(q2R)*((3148506117433717*cos(q1R))/4503599627370496 + (1211728953682539*sin(q1R))/2251799813685248))/340282366920938463463374607431768211456 - (81129635049124235038645691064225*cos(q3R)*((10914283902180054573281797610715*cos(q1R))/20282409603651670423947251286016 - (28359221366286827792295350160645*sin(q1R))/40564819207303340847894502572032))/81129638414606681695789005144064 + (2115063383689692319117831580025*sin(q3R)*((10914283902180054573281797610715*cos(q1R))/20282409603651670423947251286016 - (28359221366286827792295350160645*sin(q1R))/40564819207303340847894502572032))/10384593717069655257060992658440192 + (234819211581865*cos(q3R)*(cos(q2R)*((3148506117433717*cos(q1R))/4503599627370496 + (1211728953682539*sin(q1R))/2251799813685248) - (7514214926474921*sin(q2R)*((1211728953682539*cos(q1R))/2251799813685248 - (3148506117433717*sin(q1R))/4503599627370496))/36893488147419103232))/1152921504606846976 - (67682029681889335677290557259385*cos(q3R)*((7514214926474921*cos(q2R)*((1211728953682539*cos(q1R))/2251799813685248 - (3148506117433717*sin(q1R))/4503599627370496))/36893488147419103232 + sin(q2R)*((3148506117433717*cos(q1R))/4503599627370496 + (1211728953682539*sin(q1R))/2251799813685248)))/332306998946228968225951765070086144 + (9007199067919185*sin(q3R)*(cos(q2R)*((3148506117433717*cos(q1R))/4503599627370496 + (1211728953682539*sin(q1R))/2251799813685248) - (7514214926474921*sin(q2R)*((1211728953682539*cos(q1R))/2251799813685248 - (3148506117433717*sin(q1R))/4503599627370496))/36893488147419103232))/9007199254740992 + (1764482024691522628700660907665*sin(q3R)*((7514214926474921*cos(q2R)*((1211728953682539*cos(q1R))/2251799813685248 - (3148506117433717*sin(q1R))/4503599627370496))/36893488147419103232 + sin(q2R)*((3148506117433717*cos(q1R))/4503599627370496 + (1211728953682539*sin(q1R))/2251799813685248)))/42535295865117307932921825928971026432))/9007199254740992 + sin(q5R)*(((7514214926474921*cos(q4R))/36893488147419103232 + (4503599440548691*sin(q4R))/4503599627370496)*((9007199067919185*sin(q3R)*((10914283902180054573281797610715*cos(q1R))/20282409603651670423947251286016 - (28359221366286827792295350160645*sin(q1R))/40564819207303340847894502572032))/9007199254740992 + cos(q3R)*(cos(q2R)*((3148506117433717*cos(q1R))/4503599627370496 + (1211728953682539*sin(q1R))/2251799813685248) - (7514214926474921*sin(q2R)*((1211728953682539*cos(q1R))/2251799813685248 - (3148506117433717*sin(q1R))/4503599627370496))/36893488147419103232) + (7514214926474921*sin(q3R)*((7514214926474921*cos(q2R)*((1211728953682539*cos(q1R))/2251799813685248 - (3148506117433717*sin(q1R))/4503599627370496))/36893488147419103232 + sin(q2R)*((3148506117433717*cos(q1R))/4503599627370496 + (1211728953682539*sin(q1R))/2251799813685248)))/36893488147419103232) + ((9007199067919185*cos(q4R))/9007199254740992 - (234819211581865*sin(q4R))/1152921504606846976)*((213097284493758984364555654519459856780913684045*sin(q1R))/1496577676626844588240573268701473812127674924007424 - (82012275009546312639155898108543355135168378515*cos(q1R))/748288838313422294120286634350736906063837462003712 + (67682029681889335677290557259385*cos(q2R)*((1211728953682539*cos(q1R))/2251799813685248 - (3148506117433717*sin(q1R))/4503599627370496))/332306998946228968225951765070086144 + (9007199067919185*sin(q2R)*((3148506117433717*cos(q1R))/4503599627370496 + (1211728953682539*sin(q1R))/2251799813685248))/9007199254740992) + (7514214926474921*sin(q4R)*((9007199067919185*cos(q3R)*((10914283902180054573281797610715*cos(q1R))/20282409603651670423947251286016 - (28359221366286827792295350160645*sin(q1R))/40564819207303340847894502572032))/9007199254740992 + (7514214926474921*cos(q3R)*((7514214926474921*cos(q2R)*((1211728953682539*cos(q1R))/2251799813685248 - (3148506117433717*sin(q1R))/4503599627370496))/36893488147419103232 + sin(q2R)*((3148506117433717*cos(q1R))/4503599627370496 + (1211728953682539*sin(q1R))/2251799813685248)))/36893488147419103232 - sin(q3R)*(cos(q2R)*((3148506117433717*cos(q1R))/4503599627370496 + (1211728953682539*sin(q1R))/2251799813685248) - (7514214926474921*sin(q2R)*((1211728953682539*cos(q1R))/2251799813685248 - (3148506117433717*sin(q1R))/4503599627370496))/36893488147419103232)))/36893488147419103232)))/36893488147419103232000 + (807520961047489018778067709720399904923771262077295170375712179706208528987338271217011451790113918662491539890779991*cos(q2R)*((1211728953682539*cos(q1R))/2251799813685248 - (3148506117433717*sin(q1R))/4503599627370496))/15760802478557791684911616040057445522031895708186178667179317361698288708598884244565706501953966256322651196122726400000 + (3*cos(q2R)*((3148506117433717*cos(q1R))/4503599627370496 + (1211728953682539*sin(q1R))/2251799813685248))/100 - (712008244765680093343103025701132101054572137019*cos(q5R)*(((4503599440548691*cos(q4R))/4503599627370496 - (7514214926474921*sin(q4R))/36893488147419103232)*((9007199067919185*sin(q3R)*((10914283902180054573281797610715*cos(q1R))/20282409603651670423947251286016 - (28359221366286827792295350160645*sin(q1R))/40564819207303340847894502572032))/9007199254740992 + cos(q3R)*(cos(q2R)*((3148506117433717*cos(q1R))/4503599627370496 + (1211728953682539*sin(q1R))/2251799813685248) - (7514214926474921*sin(q2R)*((1211728953682539*cos(q1R))/2251799813685248 - (3148506117433717*sin(q1R))/4503599627370496))/36893488147419103232) + (7514214926474921*sin(q3R)*((7514214926474921*cos(q2R)*((1211728953682539*cos(q1R))/2251799813685248 - (3148506117433717*sin(q1R))/4503599627370496))/36893488147419103232 + sin(q2R)*((3148506117433717*cos(q1R))/4503599627370496 + (1211728953682539*sin(q1R))/2251799813685248)))/36893488147419103232) - ((234819211581865*cos(q4R))/1152921504606846976 + (9007199067919185*sin(q4R))/9007199254740992)*((213097284493758984364555654519459856780913684045*sin(q1R))/1496577676626844588240573268701473812127674924007424 - (82012275009546312639155898108543355135168378515*cos(q1R))/748288838313422294120286634350736906063837462003712 + (67682029681889335677290557259385*cos(q2R)*((1211728953682539*cos(q1R))/2251799813685248 - (3148506117433717*sin(q1R))/4503599627370496))/332306998946228968225951765070086144 + (9007199067919185*sin(q2R)*((3148506117433717*cos(q1R))/4503599627370496 + (1211728953682539*sin(q1R))/2251799813685248))/9007199254740992) + (7514214926474921*cos(q4R)*((9007199067919185*cos(q3R)*((10914283902180054573281797610715*cos(q1R))/20282409603651670423947251286016 - (28359221366286827792295350160645*sin(q1R))/40564819207303340847894502572032))/9007199254740992 + (7514214926474921*cos(q3R)*((7514214926474921*cos(q2R)*((1211728953682539*cos(q1R))/2251799813685248 - (3148506117433717*sin(q1R))/4503599627370496))/36893488147419103232 + sin(q2R)*((3148506117433717*cos(q1R))/4503599627370496 + (1211728953682539*sin(q1R))/2251799813685248)))/36893488147419103232 - sin(q3R)*(cos(q2R)*((3148506117433717*cos(q1R))/4503599627370496 + (1211728953682539*sin(q1R))/2251799813685248) - (7514214926474921*sin(q2R)*((1211728953682539*cos(q1R))/2251799813685248 - (3148506117433717*sin(q1R))/4503599627370496))/36893488147419103232)))/36893488147419103232))/2451992865385422173373355243440494693789982595493763481600 + (170695144106365826517608855445768431563113584343*cos(q5R)*((128527577967104929471702655059245076724477257328642562920515125*cos(q1R))/28269553036454149273332760011886696253239742350009903329945699220681916416 - (333960713126929533372903469589741180908441336378844163830032875*sin(q1R))/56539106072908298546665520023773392506479484700019806659891398441363832832 - (106069577339469832923929692356850887620017617375*cos(q2R)*((1211728953682539*cos(q1R))/2251799813685248 - (3148506117433717*sin(q1R))/4503599627370496))/12554203470773361527671578846415332832204710888928069025792 - (14115856197532180673579726082375*sin(q2R)*((3148506117433717*cos(q1R))/4503599627370496 + (1211728953682539*sin(q1R))/2251799813685248))/340282366920938463463374607431768211456 - (81129635049124235038645691064225*cos(q3R)*((10914283902180054573281797610715*cos(q1R))/20282409603651670423947251286016 - (28359221366286827792295350160645*sin(q1R))/40564819207303340847894502572032))/81129638414606681695789005144064 + (2115063383689692319117831580025*sin(q3R)*((10914283902180054573281797610715*cos(q1R))/20282409603651670423947251286016 - (28359221366286827792295350160645*sin(q1R))/40564819207303340847894502572032))/10384593717069655257060992658440192 + (234819211581865*cos(q3R)*(cos(q2R)*((3148506117433717*cos(q1R))/4503599627370496 + (1211728953682539*sin(q1R))/2251799813685248) - (7514214926474921*sin(q2R)*((1211728953682539*cos(q1R))/2251799813685248 - (3148506117433717*sin(q1R))/4503599627370496))/36893488147419103232))/1152921504606846976 - (67682029681889335677290557259385*cos(q3R)*((7514214926474921*cos(q2R)*((1211728953682539*cos(q1R))/2251799813685248 - (3148506117433717*sin(q1R))/4503599627370496))/36893488147419103232 + sin(q2R)*((3148506117433717*cos(q1R))/4503599627370496 + (1211728953682539*sin(q1R))/2251799813685248)))/332306998946228968225951765070086144 + (9007199067919185*sin(q3R)*(cos(q2R)*((3148506117433717*cos(q1R))/4503599627370496 + (1211728953682539*sin(q1R))/2251799813685248) - (7514214926474921*sin(q2R)*((1211728953682539*cos(q1R))/2251799813685248 - (3148506117433717*sin(q1R))/4503599627370496))/36893488147419103232))/9007199254740992 + (1764482024691522628700660907665*sin(q3R)*((7514214926474921*cos(q2R)*((1211728953682539*cos(q1R))/2251799813685248 - (3148506117433717*sin(q1R))/4503599627370496))/36893488147419103232 + sin(q2R)*((3148506117433717*cos(q1R))/4503599627370496 + (1211728953682539*sin(q1R))/2251799813685248)))/42535295865117307932921825928971026432))/119726214130147567059245861496117904970213993920593920 - (324259171862923063*sin(q6R)*(cos(q5R)*(((7514214926474921*cos(q4R))/36893488147419103232 + (4503599440548691*sin(q4R))/4503599627370496)*((9007199067919185*sin(q3R)*((10914283902180054573281797610715*cos(q1R))/20282409603651670423947251286016 - (28359221366286827792295350160645*sin(q1R))/40564819207303340847894502572032))/9007199254740992 + cos(q3R)*(cos(q2R)*((3148506117433717*cos(q1R))/4503599627370496 + (1211728953682539*sin(q1R))/2251799813685248) - (7514214926474921*sin(q2R)*((1211728953682539*cos(q1R))/2251799813685248 - (3148506117433717*sin(q1R))/4503599627370496))/36893488147419103232) + (7514214926474921*sin(q3R)*((7514214926474921*cos(q2R)*((1211728953682539*cos(q1R))/2251799813685248 - (3148506117433717*sin(q1R))/4503599627370496))/36893488147419103232 + sin(q2R)*((3148506117433717*cos(q1R))/4503599627370496 + (1211728953682539*sin(q1R))/2251799813685248)))/36893488147419103232) + ((9007199067919185*cos(q4R))/9007199254740992 - (234819211581865*sin(q4R))/1152921504606846976)*((213097284493758984364555654519459856780913684045*sin(q1R))/1496577676626844588240573268701473812127674924007424 - (82012275009546312639155898108543355135168378515*cos(q1R))/748288838313422294120286634350736906063837462003712 + (67682029681889335677290557259385*cos(q2R)*((1211728953682539*cos(q1R))/2251799813685248 - (3148506117433717*sin(q1R))/4503599627370496))/332306998946228968225951765070086144 + (9007199067919185*sin(q2R)*((3148506117433717*cos(q1R))/4503599627370496 + (1211728953682539*sin(q1R))/2251799813685248))/9007199254740992) + (7514214926474921*sin(q4R)*((9007199067919185*cos(q3R)*((10914283902180054573281797610715*cos(q1R))/20282409603651670423947251286016 - (28359221366286827792295350160645*sin(q1R))/40564819207303340847894502572032))/9007199254740992 + (7514214926474921*cos(q3R)*((7514214926474921*cos(q2R)*((1211728953682539*cos(q1R))/2251799813685248 - (3148506117433717*sin(q1R))/4503599627370496))/36893488147419103232 + sin(q2R)*((3148506117433717*cos(q1R))/4503599627370496 + (1211728953682539*sin(q1R))/2251799813685248)))/36893488147419103232 - sin(q3R)*(cos(q2R)*((3148506117433717*cos(q1R))/4503599627370496 + (1211728953682539*sin(q1R))/2251799813685248) - (7514214926474921*sin(q2R)*((1211728953682539*cos(q1R))/2251799813685248 - (3148506117433717*sin(q1R))/4503599627370496))/36893488147419103232)))/36893488147419103232) - (7514214926474921*sin(q5R)*(((4503599440548691*cos(q4R))/4503599627370496 - (7514214926474921*sin(q4R))/36893488147419103232)*((9007199067919185*sin(q3R)*((10914283902180054573281797610715*cos(q1R))/20282409603651670423947251286016 - (28359221366286827792295350160645*sin(q1R))/40564819207303340847894502572032))/9007199254740992 + cos(q3R)*(cos(q2R)*((3148506117433717*cos(q1R))/4503599627370496 + (1211728953682539*sin(q1R))/2251799813685248) - (7514214926474921*sin(q2R)*((1211728953682539*cos(q1R))/2251799813685248 - (3148506117433717*sin(q1R))/4503599627370496))/36893488147419103232) + (7514214926474921*sin(q3R)*((7514214926474921*cos(q2R)*((1211728953682539*cos(q1R))/2251799813685248 - (3148506117433717*sin(q1R))/4503599627370496))/36893488147419103232 + sin(q2R)*((3148506117433717*cos(q1R))/4503599627370496 + (1211728953682539*sin(q1R))/2251799813685248)))/36893488147419103232) - ((234819211581865*cos(q4R))/1152921504606846976 + (9007199067919185*sin(q4R))/9007199254740992)*((213097284493758984364555654519459856780913684045*sin(q1R))/1496577676626844588240573268701473812127674924007424 - (82012275009546312639155898108543355135168378515*cos(q1R))/748288838313422294120286634350736906063837462003712 + (67682029681889335677290557259385*cos(q2R)*((1211728953682539*cos(q1R))/2251799813685248 - (3148506117433717*sin(q1R))/4503599627370496))/332306998946228968225951765070086144 + (9007199067919185*sin(q2R)*((3148506117433717*cos(q1R))/4503599627370496 + (1211728953682539*sin(q1R))/2251799813685248))/9007199254740992) + (7514214926474921*cos(q4R)*((9007199067919185*cos(q3R)*((10914283902180054573281797610715*cos(q1R))/20282409603651670423947251286016 - (28359221366286827792295350160645*sin(q1R))/40564819207303340847894502572032))/9007199254740992 + (7514214926474921*cos(q3R)*((7514214926474921*cos(q2R)*((1211728953682539*cos(q1R))/2251799813685248 - (3148506117433717*sin(q1R))/4503599627370496))/36893488147419103232 + sin(q2R)*((3148506117433717*cos(q1R))/4503599627370496 + (1211728953682539*sin(q1R))/2251799813685248)))/36893488147419103232 - sin(q3R)*(cos(q2R)*((3148506117433717*cos(q1R))/4503599627370496 + (1211728953682539*sin(q1R))/2251799813685248) - (7514214926474921*sin(q2R)*((1211728953682539*cos(q1R))/2251799813685248 - (3148506117433717*sin(q1R))/4503599627370496))/36893488147419103232)))/36893488147419103232))/36893488147419103232 + (9007199067919185*sin(q5R)*((128527577967104929471702655059245076724477257328642562920515125*cos(q1R))/28269553036454149273332760011886696253239742350009903329945699220681916416 - (333960713126929533372903469589741180908441336378844163830032875*sin(q1R))/56539106072908298546665520023773392506479484700019806659891398441363832832 - (106069577339469832923929692356850887620017617375*cos(q2R)*((1211728953682539*cos(q1R))/2251799813685248 - (3148506117433717*sin(q1R))/4503599627370496))/12554203470773361527671578846415332832204710888928069025792 - (14115856197532180673579726082375*sin(q2R)*((3148506117433717*cos(q1R))/4503599627370496 + (1211728953682539*sin(q1R))/2251799813685248))/340282366920938463463374607431768211456 - (81129635049124235038645691064225*cos(q3R)*((10914283902180054573281797610715*cos(q1R))/20282409603651670423947251286016 - (28359221366286827792295350160645*sin(q1R))/40564819207303340847894502572032))/81129638414606681695789005144064 + (2115063383689692319117831580025*sin(q3R)*((10914283902180054573281797610715*cos(q1R))/20282409603651670423947251286016 - (28359221366286827792295350160645*sin(q1R))/40564819207303340847894502572032))/10384593717069655257060992658440192 + (234819211581865*cos(q3R)*(cos(q2R)*((3148506117433717*cos(q1R))/4503599627370496 + (1211728953682539*sin(q1R))/2251799813685248) - (7514214926474921*sin(q2R)*((1211728953682539*cos(q1R))/2251799813685248 - (3148506117433717*sin(q1R))/4503599627370496))/36893488147419103232))/1152921504606846976 - (67682029681889335677290557259385*cos(q3R)*((7514214926474921*cos(q2R)*((1211728953682539*cos(q1R))/2251799813685248 - (3148506117433717*sin(q1R))/4503599627370496))/36893488147419103232 + sin(q2R)*((3148506117433717*cos(q1R))/4503599627370496 + (1211728953682539*sin(q1R))/2251799813685248)))/332306998946228968225951765070086144 + (9007199067919185*sin(q3R)*(cos(q2R)*((3148506117433717*cos(q1R))/4503599627370496 + (1211728953682539*sin(q1R))/2251799813685248) - (7514214926474921*sin(q2R)*((1211728953682539*cos(q1R))/2251799813685248 - (3148506117433717*sin(q1R))/4503599627370496))/36893488147419103232))/9007199254740992 + (1764482024691522628700660907665*sin(q3R)*((7514214926474921*cos(q2R)*((1211728953682539*cos(q1R))/2251799813685248 - (3148506117433717*sin(q1R))/4503599627370496))/36893488147419103232 + sin(q2R)*((3148506117433717*cos(q1R))/4503599627370496 + (1211728953682539*sin(q1R))/2251799813685248)))/42535295865117307932921825928971026432))/9007199254740992))/9007199254740992000 - (22542644779424763*sin(q2R)*((1211728953682539*cos(q1R))/2251799813685248 - (3148506117433717*sin(q1R))/4503599627370496))/3689348814741910323200 + (107465779053290185796889472867275736954369330186921663479979246519176992895505610212310958309481948671*sin(q2R)*((3148506117433717*cos(q1R))/4503599627370496 + (1211728953682539*sin(q1R))/2251799813685248))/427197407184182016479004341233910422920540904471330553989408321564443945156128110004592417387315200000 - (27*cos(q5R)*(((7514214926474921*cos(q4R))/36893488147419103232 + (4503599440548691*sin(q4R))/4503599627370496)*((9007199067919185*sin(q3R)*((10914283902180054573281797610715*cos(q1R))/20282409603651670423947251286016 - (28359221366286827792295350160645*sin(q1R))/40564819207303340847894502572032))/9007199254740992 + cos(q3R)*(cos(q2R)*((3148506117433717*cos(q1R))/4503599627370496 + (1211728953682539*sin(q1R))/2251799813685248) - (7514214926474921*sin(q2R)*((1211728953682539*cos(q1R))/2251799813685248 - (3148506117433717*sin(q1R))/4503599627370496))/36893488147419103232) + (7514214926474921*sin(q3R)*((7514214926474921*cos(q2R)*((1211728953682539*cos(q1R))/2251799813685248 - (3148506117433717*sin(q1R))/4503599627370496))/36893488147419103232 + sin(q2R)*((3148506117433717*cos(q1R))/4503599627370496 + (1211728953682539*sin(q1R))/2251799813685248)))/36893488147419103232) + ((9007199067919185*cos(q4R))/9007199254740992 - (234819211581865*sin(q4R))/1152921504606846976)*((213097284493758984364555654519459856780913684045*sin(q1R))/1496577676626844588240573268701473812127674924007424 - (82012275009546312639155898108543355135168378515*cos(q1R))/748288838313422294120286634350736906063837462003712 + (67682029681889335677290557259385*cos(q2R)*((1211728953682539*cos(q1R))/2251799813685248 - (3148506117433717*sin(q1R))/4503599627370496))/332306998946228968225951765070086144 + (9007199067919185*sin(q2R)*((3148506117433717*cos(q1R))/4503599627370496 + (1211728953682539*sin(q1R))/2251799813685248))/9007199254740992) + (7514214926474921*sin(q4R)*((9007199067919185*cos(q3R)*((10914283902180054573281797610715*cos(q1R))/20282409603651670423947251286016 - (28359221366286827792295350160645*sin(q1R))/40564819207303340847894502572032))/9007199254740992 + (7514214926474921*cos(q3R)*((7514214926474921*cos(q2R)*((1211728953682539*cos(q1R))/2251799813685248 - (3148506117433717*sin(q1R))/4503599627370496))/36893488147419103232 + sin(q2R)*((3148506117433717*cos(q1R))/4503599627370496 + (1211728953682539*sin(q1R))/2251799813685248)))/36893488147419103232 - sin(q3R)*(cos(q2R)*((3148506117433717*cos(q1R))/4503599627370496 + (1211728953682539*sin(q1R))/2251799813685248) - (7514214926474921*sin(q2R)*((1211728953682539*cos(q1R))/2251799813685248 - (3148506117433717*sin(q1R))/4503599627370496))/36893488147419103232)))/36893488147419103232))/1000 + (202883803014822867*sin(q5R)*(((4503599440548691*cos(q4R))/4503599627370496 - (7514214926474921*sin(q4R))/36893488147419103232)*((9007199067919185*sin(q3R)*((10914283902180054573281797610715*cos(q1R))/20282409603651670423947251286016 - (28359221366286827792295350160645*sin(q1R))/40564819207303340847894502572032))/9007199254740992 + cos(q3R)*(cos(q2R)*((3148506117433717*cos(q1R))/4503599627370496 + (1211728953682539*sin(q1R))/2251799813685248) - (7514214926474921*sin(q2R)*((1211728953682539*cos(q1R))/2251799813685248 - (3148506117433717*sin(q1R))/4503599627370496))/36893488147419103232) + (7514214926474921*sin(q3R)*((7514214926474921*cos(q2R)*((1211728953682539*cos(q1R))/2251799813685248 - (3148506117433717*sin(q1R))/4503599627370496))/36893488147419103232 + sin(q2R)*((3148506117433717*cos(q1R))/4503599627370496 + (1211728953682539*sin(q1R))/2251799813685248)))/36893488147419103232) - ((234819211581865*cos(q4R))/1152921504606846976 + (9007199067919185*sin(q4R))/9007199254740992)*((213097284493758984364555654519459856780913684045*sin(q1R))/1496577676626844588240573268701473812127674924007424 - (82012275009546312639155898108543355135168378515*cos(q1R))/748288838313422294120286634350736906063837462003712 + (67682029681889335677290557259385*cos(q2R)*((1211728953682539*cos(q1R))/2251799813685248 - (3148506117433717*sin(q1R))/4503599627370496))/332306998946228968225951765070086144 + (9007199067919185*sin(q2R)*((3148506117433717*cos(q1R))/4503599627370496 + (1211728953682539*sin(q1R))/2251799813685248))/9007199254740992) + (7514214926474921*cos(q4R)*((9007199067919185*cos(q3R)*((10914283902180054573281797610715*cos(q1R))/20282409603651670423947251286016 - (28359221366286827792295350160645*sin(q1R))/40564819207303340847894502572032))/9007199254740992 + (7514214926474921*cos(q3R)*((7514214926474921*cos(q2R)*((1211728953682539*cos(q1R))/2251799813685248 - (3148506117433717*sin(q1R))/4503599627370496))/36893488147419103232 + sin(q2R)*((3148506117433717*cos(q1R))/4503599627370496 + (1211728953682539*sin(q1R))/2251799813685248)))/36893488147419103232 - sin(q3R)*(cos(q2R)*((3148506117433717*cos(q1R))/4503599627370496 + (1211728953682539*sin(q1R))/2251799813685248) - (7514214926474921*sin(q2R)*((1211728953682539*cos(q1R))/2251799813685248 - (3148506117433717*sin(q1R))/4503599627370496))/36893488147419103232)))/36893488147419103232))/36893488147419103232000 - (48638874966763599*sin(q5R)*((128527577967104929471702655059245076724477257328642562920515125*cos(q1R))/28269553036454149273332760011886696253239742350009903329945699220681916416 - (333960713126929533372903469589741180908441336378844163830032875*sin(q1R))/56539106072908298546665520023773392506479484700019806659891398441363832832 - (106069577339469832923929692356850887620017617375*cos(q2R)*((1211728953682539*cos(q1R))/2251799813685248 - (3148506117433717*sin(q1R))/4503599627370496))/12554203470773361527671578846415332832204710888928069025792 - (14115856197532180673579726082375*sin(q2R)*((3148506117433717*cos(q1R))/4503599627370496 + (1211728953682539*sin(q1R))/2251799813685248))/340282366920938463463374607431768211456 - (81129635049124235038645691064225*cos(q3R)*((10914283902180054573281797610715*cos(q1R))/20282409603651670423947251286016 - (28359221366286827792295350160645*sin(q1R))/40564819207303340847894502572032))/81129638414606681695789005144064 + (2115063383689692319117831580025*sin(q3R)*((10914283902180054573281797610715*cos(q1R))/20282409603651670423947251286016 - (28359221366286827792295350160645*sin(q1R))/40564819207303340847894502572032))/10384593717069655257060992658440192 + (234819211581865*cos(q3R)*(cos(q2R)*((3148506117433717*cos(q1R))/4503599627370496 + (1211728953682539*sin(q1R))/2251799813685248) - (7514214926474921*sin(q2R)*((1211728953682539*cos(q1R))/2251799813685248 - (3148506117433717*sin(q1R))/4503599627370496))/36893488147419103232))/1152921504606846976 - (67682029681889335677290557259385*cos(q3R)*((7514214926474921*cos(q2R)*((1211728953682539*cos(q1R))/2251799813685248 - (3148506117433717*sin(q1R))/4503599627370496))/36893488147419103232 + sin(q2R)*((3148506117433717*cos(q1R))/4503599627370496 + (1211728953682539*sin(q1R))/2251799813685248)))/332306998946228968225951765070086144 + (9007199067919185*sin(q3R)*(cos(q2R)*((3148506117433717*cos(q1R))/4503599627370496 + (1211728953682539*sin(q1R))/2251799813685248) - (7514214926474921*sin(q2R)*((1211728953682539*cos(q1R))/2251799813685248 - (3148506117433717*sin(q1R))/4503599627370496))/36893488147419103232))/9007199254740992 + (1764482024691522628700660907665*sin(q3R)*((7514214926474921*cos(q2R)*((1211728953682539*cos(q1R))/2251799813685248 - 